simulink model "Barriere_fermeture_geometrique_2016a"  (R2016b)
settings: Solver=VariableStepAuto  StartTime=0.0  StopTime=10.0  RelTol=1e-3
PreLoadFcn:
  | addpath('Simscape')
model workspace (MATLAB code in the model file):
  | % Simscape(TM) Multibody(TM) version: 7.0
  | 
  | % This is a model data file derived from a Simscape Multibody Import XML file using the smimport function.
  | % The data in this file sets the block parameter values in an imported Simscape Multibody model.
  | % For more information on this file, see the smimport function help page in the Simscape Multibody documentation.
  | % You can modify numerical values, but avoid any other changes to this file.
  | % Do not add code to this file. Do not edit the physical units shown in comments.
  | 
  | %%%VariableName:smiData
  | 
  | 
  | %============= RigidTransform =============%
  | 
  | %Initialize the RigidTransform structure array by filling in null values.
  | smiData.RigidTransform(115).translation = [0.0 0.0 0.0];
  | smiData.RigidTransform(115).angle = 0.0;
  | smiData.RigidTransform(115).axis = [0.0 0.0 0.0];
  | smiData.RigidTransform(115).ID = '';
  | 
  | %Translation Method - Cartesian
  | %Rotation Method - Arbitrary Axis
  | smiData.RigidTransform(1).translation = [0 0 0];  % mm
  | smiData.RigidTransform(1).angle = 0;  % rad
  | smiData.RigidTransform(1).axis = [0 0 0];
  | smiData.RigidTransform(1).ID = 'B[Bati-1:-:]';
  | 
  | %Translation Method - Cartesian
  | %Rotation Method - Arbitrary Axis
  | smiData.RigidTransform(2).translation = [0 0 0];  % mm
  | smiData.RigidTransform(2).angle = 0;  % rad
  | smiData.RigidTransform(2).axis = [0 0 0];
  | smiData.RigidTransform(2).ID = 'F[Bati-1:-:]';
  | 
  | %Translation Method - Cartesian
  | %Rotation Method - Arbitrary Axis
  | smiData.RigidTransform(3).translation = [-1.4921397450962104e-13 -2.1187831252329945e-13 201.81368327358359];  % mm
  | smiData.RigidTransform(3).angle = 2.0943951023931962;  % rad
  | smiData.RigidTransform(3).axis = [0.57735026918962606 -0.57735026918962595 0.5773502691896254];
  | smiData.RigidTransform(3).ID = 'B[Bati-1:-:Manivelle-1]';
  | 
  | %Translation Method - Cartesian
  | %Rotation Method - Arbitrary Axis
  | smiData.RigidTransform(4).translation = [-1.4110480386564174e-11 -34.999999999999446 1.9203073623444143e-11];  % mm
  | smiData.RigidTransform(4).angle = 2.0943951023931944;  % rad
  | smiData.RigidTransform(4).axis = [-0.57735026918962551 -0.57735026918962451 -0.57735026918962729];
  | smiData.RigidTransform(4).ID = 'F[Bati-1:-:Manivelle-1]';
  | 
  | %Translation Method - Cartesian
  | %Rotation Method - Arbitrary Axis
  | smiData.RigidTransform(5).translation = [79.008796978564504 9.0000000000000036 -5.500000000000286];  % mm
  | smiData.RigidTransform(5).angle = 2.0943951023931966;  % rad
  | smiData.RigidTransform(5).axis = [0.57735026918962606 -0.57735026918962595 0.57735026918962529];
  | smiData.RigidTransform(5).ID = 'B[Manivelle-1:-:Roue-1]';
  | 
  | %Translation Method - Cartesian
  | %Rotation Method - Arbitrary Axis
  | smiData.RigidTransform(6).translation = [1.0096423697092405e-11 1.4694134797821334e-11 -1.0000000000000713];  % mm
  | smiData.RigidTransform(6).angle = 3.1415926535897931;  % rad
  | smiData.RigidTransform(6).axis = [1 -3.6232584844029224e-34 -2.1942087839562885e-16];
  | smiData.RigidTransform(6).ID = 'F[Manivelle-1:-:Roue-1]';
  | 
  | %Translation Method - Cartesian
  | %Rotation Method - Arbitrary Axis
  | smiData.RigidTransform(7).translation = [2.4950194972320238e-13 126.79563556224846 92.813683273583734];  % mm
  | smiData.RigidTransform(7).angle = 2.0943951023931962;  % rad
  | smiData.RigidTransform(7).axis = [0.57735026918962606 -0.57735026918962529 0.57735026918962606];
  | smiData.RigidTransform(7).ID = 'B[Bati-1:-:Bielle-1]';
  | 
  | %Translation Method - Cartesian
  | %Rotation Method - Arbitrary Axis
  | smiData.RigidTransform(8).translation = [-1.33896240562668e-12 -185.69563556224858 1.7011796269739942e-14];  % mm
  | smiData.RigidTransform(8).angle = 2.0943951023931962;  % rad
  | smiData.RigidTransform(8).axis = [-0.57735026918962606 -0.57735026918962606 -0.57735026918962529];
  | smiData.RigidTransform(8).ID = 'F[Bati-1:-:Bielle-1]';
  | 
  | %Translation Method - Cartesian
  | %Rotation Method - Arbitrary Axis
  | smiData.RigidTransform(9).translation = [-132.59544790787075 -8.5265128291212022e-14 146.46653950343381];  % mm
  | smiData.RigidTransform(9).angle = 3.1415926535897931;  % rad
  | smiData.RigidTransform(9).axis = [-0.92883739768533258 -1.4174241145510651e-17 0.37048763631346637];
  | smiData.RigidTransform(9).ID = 'B[Bielle-1:-:Roue-1]';
  | 
  | %Translation Method - Cartesian
  | %Rotation Method - Arbitrary Axis
  | smiData.RigidTransform(10).translation = [-73.757110325617248 103.72960409807774 13.900000000000148];  % mm
  | smiData.RigidTransform(10).angle = 1.8341255936563658;  % rad
  | smiData.RigidTransform(10).axis = [-0.76611237185348935 0.45446222818459925 -0.45446222818459875];
  | smiData.RigidTransform(10).ID = 'F[Bielle-1:-:Roue-1]';
  | 
  | %Translation Method - Cartesian
  | %Rotation Method - Arbitrary Axis
  | smiData.RigidTransform(11).translation = [-855.00000000000057 -415.99999999999989 -2.997602166487909e-13];  % mm
  | smiData.RigidTransform(11).angle = 2.0943951023931953;  % rad
  | smiData.RigidTransform(11).axis = [0.57735026918962584 0.57735026918962562 0.57735026918962584];
  | smiData.RigidTransform(11).ID = 'B[Bielle-1:-:Masse_mobile-1]';
  | 
  | %Translation Method - Cartesian
  | %Rotation Method - Arbitrary Axis
  | smiData.RigidTransform(12).translation = [1155.7022886337502 2.6435895478936817e-14 1.7053025658242339e-13];  % mm
  | smiData.RigidTransform(12).angle = 2.0943951023931953;  % rad
  | smiData.RigidTransform(12).axis = [-0.57735026918962584 -0.57735026918962584 0.57735026918962584];
  | smiData.RigidTransform(12).ID = 'F[Bielle-1:-:Masse_mobile-1]';
  | 
  | %Translation Method - Cartesian
  | %Rotation Method - Arbitrary Axis
  | smiData.RigidTransform(13).translation = [0 0 43.813683273583607];  % mm
  | smiData.RigidTransform(13).angle = 3.1415926535897931;  % rad
  | smiData.RigidTransform(13).axis = [0 -7.6859349917756591e-17 1];
  | smiData.RigidTransform(13).ID = 'AssemblyGround[Bati-1:3742-1]';
  | 
  | %Translation Method - Cartesian
  | %Rotation Method - Arbitrary Axis
  | smiData.RigidTransform(14).translation = [124.99999999999996 229.50000000000017 49.813683273583663];  % mm
  | smiData.RigidTransform(14).angle = 1.8025643331517374;  % rad
  | smiData.RigidTransform(14).axis = [6.4891737650865717e-17 -5.7309259263021267e-17 1];
  | smiData.RigidTransform(14).ID = 'AssemblyGround[Bati-1:eh_12-1]';
  | 
  | %Translation Method - Cartesian
  | %Rotation Method - Arbitrary Axis
  | smiData.RigidTransform(15).translation = [-175.8775777875249 210.38468501103969 136.63945712062966];  % mm
  | smiData.RigidTransform(15).angle = 1.6861590425374564;  % rad
  | smiData.RigidTransform(15).axis = [0.5173147433723283 0.79319630861479418 0.32128658902837226];
  | smiData.RigidTransform(15).ID = 'AssemblyGround[Bati-1:Moteur-1:ehfr_6-1]';
  | 
  | %Translation Method - Cartesian
  | %Rotation Method - Arbitrary Axis
  | smiData.RigidTransform(16).translation = [-194.42155942355888 175.34681984943683 174.99999999999707];  % mm
  | smiData.RigidTransform(16).angle = 1.9203799458038229;  % rad
  | smiData.RigidTransform(16).axis = [0.36625265461228562 0.28987567884942211 -0.88421212602013133];
  | smiData.RigidTransform(16).ID = 'AssemblyGround[Bati-1:Moteur-1:MOTEUR_014-1]';
  | 
  | %Translation Method - Cartesian
  | %Rotation Method - Arbitrary Axis
  | smiData.RigidTransform(17).translation = [-175.87757778752552 210.38468501103691 213.36054287936705];  % mm
  | smiData.RigidTransform(17).angle = 1.6861590425374564;  % rad
  | smiData.RigidTransform(17).axis = [0.5173147433723283 0.79319630861479418 0.32128658902837226];
  | smiData.RigidTransform(17).ID = 'AssemblyGround[Bati-1:Moteur-1:ehfr_6-2]';
  | 
  | %Translation Method - Cartesian
  | %Rotation Method - Arbitrary Axis
  | smiData.RigidTransform(18).translation = [-193.50030490480947 135.71498239378184 213.36054287937054];  % mm
  | smiData.RigidTransform(18).angle = 1.5798154611582129;  % rad
  | smiData.RigidTransform(18).axis = [0.13562103621123053 0.98623959459989585 -0.094543093774347442];
  | smiData.RigidTransform(18).ID = 'AssemblyGround[Bati-1:Moteur-1:ehfr_6-3]';
  | 
  | %Translation Method - Cartesian
  | %Rotation Method - Arbitrary Axis
  | smiData.RigidTransform(19).translation = [-189.50324309587222 213.6004656168802 136.63945712062966];  % mm
  | smiData.RigidTransform(19).angle = 2.682320000710968;  % rad
  | smiData.RigidTransform(19).axis = [0.61543871803223826 -0.38543093102275494 -0.68751595018426104];
  | smiData.RigidTransform(19).ID = 'AssemblyGround[Bati-1:Moteur-1:vchc_6_30-1]';
  | 
  | %Translation Method - Cartesian
  | %Rotation Method - Arbitrary Axis
  | smiData.RigidTransform(20).translation = [-207.12597021315676 138.93076299962223 136.63945712062986];  % mm
  | smiData.RigidTransform(20).angle = 2.4395162248310025;  % rad
  | smiData.RigidTransform(20).axis = [0.55627663095078395 -0.50755250127944629 -0.65798690587505093];
  | smiData.RigidTransform(20).ID = 'AssemblyGround[Bati-1:Moteur-1:vchc_6_30-2]';
  | 
  | %Translation Method - Cartesian
  | %Rotation Method - Arbitrary Axis
  | smiData.RigidTransform(21).translation = [-207.12597021315671 138.93076299962235 213.36054287937054];  % mm
  | smiData.RigidTransform(21).angle = 2.4395162248310025;  % rad
  | smiData.RigidTransform(21).axis = [0.55627663095078395 -0.50755250127944629 -0.65798690587505093];
  | smiData.RigidTransform(21).ID = 'AssemblyGround[Bati-1:Moteur-1:vchc_6_30-3]';
  | 
  | %Translation Method - Cartesian
  | %Rotation Method - Arbitrary Axis
  | smiData.RigidTransform(22).translation = [-189.50324309587285 213.60046561687741 213.36054287936705];  % mm
  | smiData.RigidTransform(22).angle = 2.4395162248310025;  % rad
  | smiData.RigidTransform(22).axis = [0.55627663095078395 -0.50755250127944629 -0.65798690587505093];
  | smiData.RigidTransform(22).ID = 'AssemblyGround[Bati-1:Moteur-1:vchc_6_30-4]';
  | 
  | %Translation Method - Cartesian
  | %Rotation Method - Arbitrary Axis
  | smiData.RigidTransform(23).translation = [-193.50030490480938 135.71498239378172 136.63945712062986];  % mm
  | smiData.RigidTransform(23).angle = 1.5798154611582129;  % rad
  | smiData.RigidTransform(23).axis = [0.13562103621123026 0.98623959459989607 -0.094543093774347456];
  | smiData.RigidTransform(23).ID = 'AssemblyGround[Bati-1:Moteur-1:ehfr_6-4]';
  | 
  | %Translation Method - Cartesian
  | %Rotation Method - Arbitrary Axis
  | smiData.RigidTransform(24).translation = [125.99999999999656 229.50000000000006 46.813683273586562];  % mm
  | smiData.RigidTransform(24).angle = 1.8025643331517369;  % rad
  | smiData.RigidTransform(24).axis = [6.3930876709235808e-17 -1.1805373058737908e-16 1];
  | smiData.RigidTransform(24).ID = 'AssemblyGround[Bati-1:Moteur-1]';
  | 
  | %Translation Method - Cartesian
  | %Rotation Method - Arbitrary Axis
  | smiData.RigidTransform(25).translation = [64.223317737885779 178.52133054270737 21.000000000000053];  % mm
  | smiData.RigidTransform(25).angle = 1.3390283204380566;  % rad
  | smiData.RigidTransform(25).axis = [1.3951389385649892e-16 -1.4208309664535837e-16 1];
  | smiData.RigidTransform(25).ID = 'AssemblyGround[Bati-1:Roulement_2-1:ehfr_14-2]';
  | 
  | %Translation Method - Cartesian
  | %Rotation Method - Arbitrary Axis
  | smiData.RigidTransform(26).translation = [64.223317737885779 178.52133054270737 19.000000000000053];  % mm
  | smiData.RigidTransform(26).angle = 1.3390283204380566;  % rad
  | smiData.RigidTransform(26).axis = [1.3951389385649892e-16 -1.4208309664535837e-16 1];
  | smiData.RigidTransform(26).ID = 'AssemblyGround[Bati-1:Roulement_2-1:rond_m_14-2]';
  | 
  | %Translation Method - Cartesian
  | %Rotation Method - Arbitrary Axis
  | smiData.RigidTransform(27).translation = [64.223317737885779 178.52133054270737 -5.9999999999999565];  % mm
  | smiData.RigidTransform(27).angle = 1.586709603785015;  % rad
  | smiData.RigidTransform(27).axis = [0.98421200917482088 -0.12515334792977473 -0.12515334792977512];
  | smiData.RigidTransform(27).ID = 'AssemblyGround[Bati-1:Roulement_2-1:VIS_TF2E_001-2]';
  | 
  | %Translation Method - Cartesian
  | %Rotation Method - Arbitrary Axis
  | smiData.RigidTransform(28).translation = [35.051593670618466 54.91708095984221 21.000000000000011];  % mm
  | smiData.RigidTransform(28).angle = 1.3390283204380566;  % rad
  | smiData.RigidTransform(28).axis = [1.3951389385649892e-16 -1.4208309664535837e-16 1];
  | smiData.RigidTransform(28).ID = 'AssemblyGround[Bati-1:Roulement_2-1:ehfr_14-1]';
  | 
  | %Translation Method - Cartesian
  | %Rotation Method - Arbitrary Axis
  | smiData.RigidTransform(29).translation = [49.637455704252211 116.719205751275 0];  % mm
  | smiData.RigidTransform(29).angle = 1.8025643331517369;  % rad
  | smiData.RigidTransform(29).axis = [9.3810881603968918e-17 2.516618558763085e-16 -1];
  | smiData.RigidTransform(29).ID = 'AssemblyGround[Bati-1:Roulement_2-1:roul_010-1]';
  | 
  | %Translation Method - Cartesian
  | %Rotation Method - Arbitrary Axis
  | smiData.RigidTransform(30).translation = [35.051593670618466 54.91708095984221 19.000000000000011];  % mm
  | smiData.RigidTransform(30).angle = 1.3390283204380566;  % rad
  | smiData.RigidTransform(30).axis = [1.3951389385649892e-16 -1.4208309664535837e-16 1];
  | smiData.RigidTransform(30).ID = 'AssemblyGround[Bati-1:Roulement_2-1:rond_m_14-1]';
  | 
  | %Translation Method - Cartesian
  | %Rotation Method - Arbitrary Axis
  | smiData.RigidTransform(31).translation = [35.051593670618466 54.917080959842238 -5.9999999999998526];  % mm
  | smiData.RigidTransform(31).angle = 1.584165821206561;  % rad
  | smiData.RigidTransform(31).axis = [0.98671908730881319 -0.11485957239268889 -0.114859572392689];
  | smiData.RigidTransform(31).ID = 'AssemblyGround[Bati-1:Roulement_2-1:VIS_TF2E_001-1]';
  | 
  | %Translation Method - Cartesian
  | %Rotation Method - Arbitrary Axis
  | smiData.RigidTransform(32).translation = [124.81984509590156 230.00190937854114 49.813683273583685];  % mm
  | smiData.RigidTransform(32).angle = 1.8025643331517369;  % rad
  | smiData.RigidTransform(32).axis = [-9.3810881603968918e-17 -2.516618558763085e-16 1];
  | smiData.RigidTransform(32).ID = 'AssemblyGround[Bati-1:Roulement_2-1]';
  | 
  | %Translation Method - Cartesian
  | %Rotation Method - Arbitrary Axis
  | smiData.RigidTransform(33).translation = [124.99999999999994 21.00000000000005 49.813683273583685];  % mm
  | smiData.RigidTransform(33).angle = 1.8025643331517374;  % rad
  | smiData.RigidTransform(33).axis = [6.4891737650865717e-17 -5.7309259263021267e-17 1];
  | smiData.RigidTransform(33).ID = 'AssemblyGround[Bati-1:eh_12-2]';
  | 
  | %Translation Method - Cartesian
  | %Rotation Method - Arbitrary Axis
  | smiData.RigidTransform(34).translation = [-125 229.50000000000017 49.813683273583656];  % mm
  | smiData.RigidTransform(34).angle = 1.8025643331517374;  % rad
  | smiData.RigidTransform(34).axis = [6.4891737650865717e-17 -5.7309259263021267e-17 1];
  | smiData.RigidTransform(34).ID = 'AssemblyGround[Bati-1:eh_12-3]';
  | 
  | %Translation Method - Cartesian
  | %Rotation Method - Arbitrary Axis
  | smiData.RigidTransform(35).translation = [-125.00000000000006 21.000000000000046 49.813683273583699];  % mm
  | smiData.RigidTransform(35).angle = 1.8025643331517374;  % rad
  | smiData.RigidTransform(35).axis = [0 0 1];
  | smiData.RigidTransform(35).ID = 'AssemblyGround[Bati-1:eh_12-4]';
  | 
  | %Translation Method - Cartesian
  | %Rotation Method - Arbitrary Axis
  | smiData.RigidTransform(36).translation = [-233.39343399959662 123.4099062712389 43.000000000000028];  % mm
  | smiData.RigidTransform(36).angle = 2.1269062011022761;  % rad
  | smiData.RigidTransform(36).axis = [-0.44439290189209107 0.67602805443717784 -0.58779334664643024];
  | smiData.RigidTransform(36).ID = 'AssemblyGround[Bati-1:Roulement_1-1:rond_m_10-2]';
  | 
  | %Translation Method - Cartesian
  | %Rotation Method - Arbitrary Axis
  | smiData.RigidTransform(37).translation = [-205.93473899471468 237.14371860789134 43.000000000000057];  % mm
  | smiData.RigidTransform(37).angle = 3.0234649588732694;  % rad
  | smiData.RigidTransform(37).axis = [-0.70057844934475677 0.10458570654058162 0.70586943998242579];
  | smiData.RigidTransform(37).ID = 'AssemblyGround[Bati-1:Roulement_1-1:vh_10_45 8-8-1]';
  | 
  | %Translation Method - Cartesian
  | %Rotation Method - Arbitrary Axis
  | smiData.RigidTransform(38).translation = [-231.44691038411835 122.9505090418331 43.000000000000028];  % mm
  | smiData.RigidTransform(38).angle = 1.8561332144596066;  % rad
  | smiData.RigidTransform(38).axis = [0.6281370768124086 0.62112083286202469 0.46867123201488148];
  | smiData.RigidTransform(38).ID = 'AssemblyGround[Bati-1:Roulement_1-1:ENTRETOISE_023-2]';
  | 
  | %Translation Method - Cartesian
  | %Rotation Method - Arbitrary Axis
  | smiData.RigidTransform(39).translation = [-204.38387611565184 176.67054418872968 43.000000000000043];  % mm
  | smiData.RigidTransform(39).angle = 2.2329912010448152;  % rad
  | smiData.RigidTransform(39).axis = [0.48837040813325044 -0.6170471393904029 -0.6170471393904059];
  | smiData.RigidTransform(39).ID = 'AssemblyGround[Bati-1:Roulement_1-1:roul_009-1]';
  | 
  | %Translation Method - Cartesian
  | %Rotation Method - Arbitrary Axis
  | smiData.RigidTransform(40).translation = [-232.80947691495311 123.27208710241713 43.000000000000028];  % mm
  | smiData.RigidTransform(40).angle = 3.0234649588732694;  % rad
  | smiData.RigidTransform(40).axis = [-0.70057844934475666 0.10458570654058141 0.70586943998242591];
  | smiData.RigidTransform(40).ID = 'AssemblyGround[Bati-1:Roulement_1-1:vh_10_45 8-8-2]';
  | 
  | %Translation Method - Cartesian
  | %Rotation Method - Arbitrary Axis
  | smiData.RigidTransform(41).translation = [-204.57217246387992 236.82214054730727 43.000000000000057];  % mm
  | smiData.RigidTransform(41).angle = 2.232991201044813;  % rad
  | smiData.RigidTransform(41).axis = [-0.48837040813324945 0.61704713939040501 -0.61704713939040456];
  | smiData.RigidTransform(41).ID = 'AssemblyGround[Bati-1:Roulement_1-1:ENTRETOISE_023-1]';
  | 
  | %Translation Method - Cartesian
  | %Rotation Method - Arbitrary Axis
  | smiData.RigidTransform(42).translation = [-202.24905615194552 116.05955060074632 43.000000000000028];  % mm
  | smiData.RigidTransform(42).angle = 1.5777653498429955;  % rad
  | smiData.RigidTransform(42).axis = [0.14713680523855655 0.98561149764352873 -0.083190962592528811];
  | smiData.RigidTransform(42).ID = 'AssemblyGround[Bati-1:Roulement_1-1:ehfr_10-2]';
  | 
  | %Translation Method - Cartesian
  | %Rotation Method - Arbitrary Axis
  | smiData.RigidTransform(43).translation = [-175.37431823170709 229.93118210622052 43.000000000000057];  % mm
  | smiData.RigidTransform(43).angle = 2.3554366301540348;  % rad
  | smiData.RigidTransform(43).axis = [-0.53100028324755 0.55137024942272572 -0.64345127806427027];
  | smiData.RigidTransform(43).ID = 'AssemblyGround[Bati-1:Roulement_1-1:ehfr_10-1]';
  | 
  | %Translation Method - Cartesian
  | %Rotation Method - Arbitrary Axis
  | smiData.RigidTransform(44).translation = [-206.51869607935814 237.28153777671307 43.000000000000057];  % mm
  | smiData.RigidTransform(44).angle = 3.1212647204710873;  % rad
  | smiData.RigidTransform(44).axis = [0.69049920252183583 -0.15252051659504276 0.70707025346445607];
  | smiData.RigidTransform(44).ID = 'AssemblyGround[Bati-1:Roulement_1-1:rond_m_10-1]';
  | 
  | %Translation Method - Cartesian
  | %Rotation Method - Arbitrary Axis
  | smiData.RigidTransform(45).translation = [125.00000000000017 229.50000000000017 49.813683273583898];  % mm
  | smiData.RigidTransform(45).angle = 1.8025643331517378;  % rad
  | smiData.RigidTransform(45).axis = [-2.9335469981929225e-16 -2.9342350937782738e-16 1];
  | smiData.RigidTransform(45).ID = 'AssemblyGround[Bati-1:Roulement_1-1]';
  | 
  | %Translation Method - Cartesian
  | %Rotation Method - Arbitrary Axis
  | smiData.RigidTransform(46).translation = [-125 229.5 43.813683273583777];  % mm
  | smiData.RigidTransform(46).angle = 3.1415926535897931;  % rad
  | smiData.RigidTransform(46).axis = [-0.98074665978199183 -0.1952843806515665 -1.3884606460031711e-16];
  | smiData.RigidTransform(46).ID = 'AssemblyGround[Bati-1:entretoise base-1]';
  | 
  | %Translation Method - Cartesian
  | %Rotation Method - Arbitrary Axis
  | smiData.RigidTransform(47).translation = [124.99999999999999 21.000000000000043 43.813683273583727];  % mm
  | smiData.RigidTransform(47).angle = 3.1415926535897931;  % rad
  | smiData.RigidTransform(47).axis = [-0.98074665978199183 -0.1952843806515665 -1.3884606460031711e-16];
  | smiData.RigidTransform(47).ID = 'AssemblyGround[Bati-1:entretoise base-4]';
  | 
  | %Translation Method - Cartesian
  | %Rotation Method - Arbitrary Axis
  | smiData.RigidTransform(48).translation = [0 0 0];  % mm
  | smiData.RigidTransform(48).angle = 1.5707963267948968;  % rad
  | smiData.RigidTransform(48).axis = [1 0 0];
  | smiData.RigidTransform(48).ID = 'AssemblyGround[Bati-1:support moteur-1]';
  | 
  | %Translation Method - Cartesian
  | %Rotation Method - Arbitrary Axis
  | smiData.RigidTransform(49).translation = [-160.0000000000004 -287.99999999999989 -10.000000000000002];  % mm
  | smiData.RigidTransform(49).angle = 2.0943951023931953;  % rad
  | smiData.RigidTransform(49).axis = [-0.57735026918962595 -0.57735026918962562 0.57735026918962562];
  | smiData.RigidTransform(49).ID = 'AssemblyGround[Bati-1:pied-1:plateau superieur-1]';
  | 
  | %Translation Method - Cartesian
  | %Rotation Method - Arbitrary Axis
  | smiData.RigidTransform(50).translation = [-125.00000000000189 -200.50000000000304 -912.9999999999925];  % mm
  | smiData.RigidTransform(50).angle = 1.5707963267948968;  % rad
  | smiData.RigidTransform(50).axis = [1 -1.6431300764452314e-14 0];
  | smiData.RigidTransform(50).ID = 'AssemblyGround[Bati-1:pied-1:base pied-1]';
  | 
  | %Translation Method - Cartesian
  | %Rotation Method - Arbitrary Axis
  | smiData.RigidTransform(51).translation = [-474.99999999997806 -300.500000000005 -920.9999999999925];  % mm
  | smiData.RigidTransform(51).angle = 1.5707963267948968;  % rad
  | smiData.RigidTransform(51).axis = [1 0 0];
  | smiData.RigidTransform(51).ID = 'AssemblyGround[Bati-1:pied-1:socle-1]';
  | 
  | %Translation Method - Cartesian
  | %Rotation Method - Arbitrary Axis
  | smiData.RigidTransform(52).translation = [-125.00000000000028 -122.50000000000315 -912.9999999999925];  % mm
  | smiData.RigidTransform(52).angle = 2.0943951023931859;  % rad
  | smiData.RigidTransform(52).axis = [0.57735026918962262 -0.57735026918963206 0.57735026918962262];
  | smiData.RigidTransform(52).ID = 'AssemblyGround[Bati-1:pied-1:renfort pied-1]';
  | 
  | %Translation Method - Cartesian
  | %Rotation Method - Arbitrary Axis
  | smiData.RigidTransform(53).translation = [0 0 43.813683273583877];  % mm
  | smiData.RigidTransform(53).angle = 3.1415926535897927;  % rad
  | smiData.RigidTransform(53).axis = [-0 -0 -1];
  | smiData.RigidTransform(53).ID = 'AssemblyGround[Bati-1:pied-1]';
  | 
  | %Translation Method - Cartesian
  | %Rotation Method - Arbitrary Axis
  | smiData.RigidTransform(54).translation = [136.49999999999997 256 -50];  % mm
  | smiData.RigidTransform(54).angle = 1.5707963267948968;  % rad
  | smiData.RigidTransform(54).axis = [1 0 0];
  | smiData.RigidTransform(54).ID = 'AssemblyGround[Bati-1:Assemblage pupitre-1:C60-1]';
  | 
  | %Translation Method - Cartesian
  | %Rotation Method - Arbitrary Axis
  | smiData.RigidTransform(55).translation = [122.00000000000001 88.999999999999972 3.5000000000000031];  % mm
  | smiData.RigidTransform(55).angle = 2.8645335361772575;  % rad
  | smiData.RigidTransform(55).axis = [0.13942256184718882 -0.70020045317322044 -0.70020045317322044];
  | smiData.RigidTransform(55).ID = 'AssemblyGround[Bati-1:Assemblage pupitre-1:douille_4mm_rouge-1]';
  | 
  | %Translation Method - Cartesian
  | %Rotation Method - Arbitrary Axis
  | smiData.RigidTransform(56).translation = [182 70 3.5000000000000031];  % mm
  | smiData.RigidTransform(56).angle = 2.8645335361772575;  % rad
  | smiData.RigidTransform(56).axis = [0.13942256184718882 -0.70020045317322044 -0.70020045317322044];
  | smiData.RigidTransform(56).ID = 'AssemblyGround[Bati-1:Assemblage pupitre-1:douille_4mm_rouge-5]';
  | 
  | %Translation Method - Cartesian
  | %Rotation Method - Arbitrary Axis
  | smiData.RigidTransform(57).translation = [102.49999999999997 110.49999999999993 10.500000000000002];  % mm
  | smiData.RigidTransform(57).angle = 0;  % rad
  | smiData.RigidTransform(57).axis = [0 0 0];
  | smiData.RigidTransform(57).ID = 'AssemblyGround[Bati-1:Assemblage pupitre-1:atv-1]';
  | 
  | %Translation Method - Cartesian
  | %Rotation Method - Arbitrary Axis
  | smiData.RigidTransform(58).translation = [152 88.999999999999972 3.5000000000000031];  % mm
  | smiData.RigidTransform(58).angle = 2.8645335361772575;  % rad
  | smiData.RigidTransform(58).axis = [0.13942256184718882 -0.70020045317322044 -0.70020045317322044];
  | smiData.RigidTransform(58).ID = 'AssemblyGround[Bati-1:Assemblage pupitre-1:douille_4mm_rouge-4]';
  | 
  | %Translation Method - Cartesian
  | %Rotation Method - Arbitrary Axis
  | smiData.RigidTransform(59).translation = [182 89.000000000000028 3.5000000000000031];  % mm
  | smiData.RigidTransform(59).angle = 2.8645335361772575;  % rad
  | smiData.RigidTransform(59).axis = [0.13942256184718882 -0.70020045317322044 -0.70020045317322044];
  | smiData.RigidTransform(59).ID = 'AssemblyGround[Bati-1:Assemblage pupitre-1:douille_4mm_rouge-2]';
  | 
  | %Translation Method - Cartesian
  | %Rotation Method - Arbitrary Axis
  | smiData.RigidTransform(60).translation = [122.00000000000003 69.999999999999957 3.5000000000000031];  % mm
  | smiData.RigidTransform(60).angle = 2.8645335361772575;  % rad
  | smiData.RigidTransform(60).axis = [0.13942256184718882 -0.70020045317322044 -0.70020045317322044];
  | smiData.RigidTransform(60).ID = 'AssemblyGround[Bati-1:Assemblage pupitre-1:douille_4mm_rouge-3]';
  | 
  | %Translation Method - Cartesian
  | %Rotation Method - Arbitrary Axis
  | smiData.RigidTransform(61).translation = [15 15 -20.000000000000018];  % mm
  | smiData.RigidTransform(61).angle = 0;  % rad
  | smiData.RigidTransform(61).axis = [0 0 0];
  | smiData.RigidTransform(61).ID = 'AssemblyGround[Bati-1:Assemblage pupitre-1:bouton_tournant_clé-1:embase_BT_clé-2]';
  | 
  | %Translation Method - Cartesian
  | %Rotation Method - Arbitrary Axis
  | smiData.RigidTransform(62).translation = [12.483450518527395 35.01481477798076 -21.990742270930674];  % mm
  | smiData.RigidTransform(62).angle = 1.0104350246787706;  % rad
  | smiData.RigidTransform(62).axis = [-0.0054592338395522983 -0.999968069200867 -0.0058358670799844572];
  | smiData.RigidTransform(62).ID = 'AssemblyGround[Bati-1:Assemblage pupitre-1:bouton_tournant_clé-1:clé-1]';
  | 
  | %Translation Method - Cartesian
  | %Rotation Method - Arbitrary Axis
  | smiData.RigidTransform(63).translation = [0 0 0];  % mm
  | smiData.RigidTransform(63).angle = 0;  % rad
  | smiData.RigidTransform(63).axis = [0 0 0];
  | smiData.RigidTransform(63).ID = 'AssemblyGround[Bati-1:Assemblage pupitre-1:bouton_tournant_clé-1:embase_BP_2_contacts-1]';
  | 
  | %Translation Method - Cartesian
  | %Rotation Method - Arbitrary Axis
  | smiData.RigidTransform(64).translation = [15 24.000000000000007 -20.000000000000018];  % mm
  | smiData.RigidTransform(64).angle = 0;  % rad
  | smiData.RigidTransform(64).axis = [0 0 0];
  | smiData.RigidTransform(64).ID = 'AssemblyGround[Bati-1:Assemblage pupitre-1:bouton_tournant_clé-1:corps_BT_clé-1]';
  | 
  | %Translation Method - Cartesian
  | %Rotation Method - Arbitrary Axis
  | smiData.RigidTransform(65).translation = [22.000000000000007 94.999999999999972 -13.500000000000012];  % mm
  | smiData.RigidTransform(65).angle = 1.5707963267948968;  % rad
  | smiData.RigidTransform(65).axis = [1 0 0];
  | smiData.RigidTransform(65).ID = 'AssemblyGround[Bati-1:Assemblage pupitre-1:bouton_tournant_clé-1]';
  | 
  | %Translation Method - Cartesian
  | %Rotation Method - Arbitrary Axis
  | smiData.RigidTransform(66).translation = [-8.0000000000000071 0 0];  % mm
  | smiData.RigidTransform(66).angle = 0;  % rad
  | smiData.RigidTransform(66).axis = [0 0 0];
  | smiData.RigidTransform(66).ID = 'AssemblyGround[Bati-1:Assemblage pupitre-1:tole mesures-1]';
  | 
  | %Translation Method - Cartesian
  | %Rotation Method - Arbitrary Axis
  | smiData.RigidTransform(67).translation = [0 0 21.999999999999993];  % mm
  | smiData.RigidTransform(67).angle = 0;  % rad
  | smiData.RigidTransform(67).axis = [0 0 0];
  | smiData.RigidTransform(67).ID = 'AssemblyGround[Bati-1:Assemblage pupitre-1:voyant_vert-1:tête_voyant_vert-1]';
  | 
  | %Translation Method - Cartesian
  | %Rotation Method - Arbitrary Axis
  | smiData.RigidTransform(68).translation = [0 0 0];  % mm
  | smiData.RigidTransform(68).angle = 0;  % rad
  | smiData.RigidTransform(68).axis = [0 0 0];
  | smiData.RigidTransform(68).ID = 'AssemblyGround[Bati-1:Assemblage pupitre-1:voyant_vert-1:corps_voyant_24V-1]';
  | 
  | %Translation Method - Cartesian
  | %Rotation Method - Arbitrary Axis
  | smiData.RigidTransform(69).translation = [37.000000000000007 305.00000000000006 -20.499999999999989];  % mm
  | smiData.RigidTransform(69).angle = 0;  % rad
  | smiData.RigidTransform(69).axis = [0 0 0];
  | smiData.RigidTransform(69).ID = 'AssemblyGround[Bati-1:Assemblage pupitre-1:voyant_vert-1]';
  | 
  | %Translation Method - Cartesian
  | %Rotation Method - Arbitrary Axis
  | smiData.RigidTransform(70).translation = [152 69.999999999999957 3.5000000000000031];  % mm
  | smiData.RigidTransform(70).angle = 2.8645335361772575;  % rad
  | smiData.RigidTransform(70).axis = [0.13942256184718882 -0.70020045317322044 -0.70020045317322044];
  | smiData.RigidTransform(70).ID = 'AssemblyGround[Bati-1:Assemblage pupitre-1:douille_4mm_rouge-6]';
  | 
  | %Translation Method - Cartesian
  | %Rotation Method - Arbitrary Axis
  | smiData.RigidTransform(71).translation = [-1.999999999999988 -17.999999999999989 24.999999999999996];  % mm
  | smiData.RigidTransform(71).angle = 0;  % rad
  | smiData.RigidTransform(71).axis = [0 0 0];
  | smiData.RigidTransform(71).ID = 'AssemblyGround[Bati-1:Assemblage pupitre-1:inter_sectionneur-1:inter_sectionneur_vario_4-1]';
  | 
  | %Translation Method - Cartesian
  | %Rotation Method - Arbitrary Axis
  | smiData.RigidTransform(72).translation = [0 0 0];  % mm
  | smiData.RigidTransform(72).angle = 0;  % rad
  | smiData.RigidTransform(72).axis = [0 0 0];
  | smiData.RigidTransform(72).ID = 'AssemblyGround[Bati-1:Assemblage pupitre-1:inter_sectionneur-1:inter_sectionneur_vario_1-1]';
  | 
  | %Translation Method - Cartesian
  | %Rotation Method - Arbitrary Axis
  | smiData.RigidTransform(73).translation = [0 0 0];  % mm
  | smiData.RigidTransform(73).angle = 0;  % rad
  | smiData.RigidTransform(73).axis = [0 0 0];
  | smiData.RigidTransform(73).ID = 'AssemblyGround[Bati-1:Assemblage pupitre-1:inter_sectionneur-1:inter_sectionneur_vario_2-1]';
  | 
  | %Translation Method - Cartesian
  | %Rotation Method - Arbitrary Axis
  | smiData.RigidTransform(74).translation = [0 0 -0.50000000000000044];  % mm
  | smiData.RigidTransform(74).angle = 0;  % rad
  | smiData.RigidTransform(74).axis = [0 0 0];
  | smiData.RigidTransform(74).ID = 'AssemblyGround[Bati-1:Assemblage pupitre-1:inter_sectionneur-1:inter_sectionneur_vario_3-1]';
  | 
  | %Translation Method - Cartesian
  | %Rotation Method - Arbitrary Axis
  | smiData.RigidTransform(75).translation = [36.999999999999993 240 1.5000000000000013];  % mm
  | smiData.RigidTransform(75).angle = 0;  % rad
  | smiData.RigidTransform(75).axis = [0 0 0];
  | smiData.RigidTransform(75).ID = 'AssemblyGround[Bati-1:Assemblage pupitre-1:inter_sectionneur-1]';
  | 
  | %Translation Method - Cartesian
  | %Rotation Method - Arbitrary Axis
  | smiData.RigidTransform(76).translation = [122.00000000000001 70 -8.4999999999999929];  % mm
  | smiData.RigidTransform(76).angle = 0;  % rad
  | smiData.RigidTransform(76).axis = [0 0 0];
  | smiData.RigidTransform(76).ID = 'AssemblyGround[Bati-1:Assemblage pupitre-1:cavalier_douille_4mm-1]';
  | 
  | %Translation Method - Cartesian
  | %Rotation Method - Arbitrary Axis
  | smiData.RigidTransform(77).translation = [182 70 -8.5];  % mm
  | smiData.RigidTransform(77).angle = 0;  % rad
  | smiData.RigidTransform(77).axis = [0 0 0];
  | smiData.RigidTransform(77).ID = 'AssemblyGround[Bati-1:Assemblage pupitre-1:cavalier_douille_4mm-2]';
  | 
  | %Translation Method - Cartesian
  | %Rotation Method - Arbitrary Axis
  | smiData.RigidTransform(78).translation = [0 0 0];  % mm
  | smiData.RigidTransform(78).angle = 0;  % rad
  | smiData.RigidTransform(78).axis = [0 0 0];
  | smiData.RigidTransform(78).ID = 'AssemblyGround[Bati-1:Assemblage pupitre-1:BP_noir-2:embase_BP_2_contacts-1]';
  | 
  | %Translation Method - Cartesian
  | %Rotation Method - Arbitrary Axis
  | smiData.RigidTransform(79).translation = [15 8.0000000000000071 -20.000000000000018];  % mm
  | smiData.RigidTransform(79).angle = 1.5707963267948968;  % rad
  | smiData.RigidTransform(79).axis = [-1 -0 -0];
  | smiData.RigidTransform(79).ID = 'AssemblyGround[Bati-1:Assemblage pupitre-1:BP_noir-2:corps_BP-3]';
  | 
  | %Translation Method - Cartesian
  | %Rotation Method - Arbitrary Axis
  | smiData.RigidTransform(80).translation = [14.999999999999986 26.000000000000021 -20.000000000000018];  % mm
  | smiData.RigidTransform(80).angle = 1.5707963267948968;  % rad
  | smiData.RigidTransform(80).axis = [-1 -0 -0];
  | smiData.RigidTransform(80).ID = 'AssemblyGround[Bati-1:Assemblage pupitre-1:BP_noir-2:tête_BP_noir-1]';
  | 
  | %Translation Method - Cartesian
  | %Rotation Method - Arbitrary Axis
  | smiData.RigidTransform(81).translation = [22.000000000000007 44.999999999999929 -20.500000000000018];  % mm
  | smiData.RigidTransform(81).angle = 1.5707963267948968;  % rad
  | smiData.RigidTransform(81).axis = [1 0 0];
  | smiData.RigidTransform(81).ID = 'AssemblyGround[Bati-1:Assemblage pupitre-1:BP_noir-2]';
  | 
  | %Translation Method - Cartesian
  | %Rotation Method - Arbitrary Axis
  | smiData.RigidTransform(82).translation = [152.00000000000003 70 -8.5];  % mm
  | smiData.RigidTransform(82).angle = 0;  % rad
  | smiData.RigidTransform(82).axis = [0 0 0];
  | smiData.RigidTransform(82).ID = 'AssemblyGround[Bati-1:Assemblage pupitre-1:cavalier_douille_4mm-3]';
  | 
  | %Translation Method - Cartesian
  | %Rotation Method - Arbitrary Axis
  | smiData.RigidTransform(83).translation = [0 0 0];  % mm
  | smiData.RigidTransform(83).angle = 0;  % rad
  | smiData.RigidTransform(83).axis = [0 0 0];
  | smiData.RigidTransform(83).ID = 'AssemblyGround[Bati-1:Assemblage pupitre-1:BP_noir-1:embase_BP_2_contacts-1]';
  | 
  | %Translation Method - Cartesian
  | %Rotation Method - Arbitrary Axis
  | smiData.RigidTransform(84).translation = [15 8.0000000000000071 -20.000000000000018];  % mm
  | smiData.RigidTransform(84).angle = 1.5707963267948968;  % rad
  | smiData.RigidTransform(84).axis = [-1 -0 -0];
  | smiData.RigidTransform(84).ID = 'AssemblyGround[Bati-1:Assemblage pupitre-1:BP_noir-1:corps_BP-3]';
  | 
  | %Translation Method - Cartesian
  | %Rotation Method - Arbitrary Axis
  | smiData.RigidTransform(85).translation = [14.999999999999986 26.000000000000021 -20.000000000000018];  % mm
  | smiData.RigidTransform(85).angle = 1.5707963267948968;  % rad
  | smiData.RigidTransform(85).axis = [-1 -0 -0];
  | smiData.RigidTransform(85).ID = 'AssemblyGround[Bati-1:Assemblage pupitre-1:BP_noir-1:tête_BP_noir-1]';
  | 
  | %Translation Method - Cartesian
  | %Rotation Method - Arbitrary Axis
  | smiData.RigidTransform(86).translation = [22.000000000000007 145.00000000000003 -20.500000000000018];  % mm
  | smiData.RigidTransform(86).angle = 1.5707963267948968;  % rad
  | smiData.RigidTransform(86).axis = [1 0 0];
  | smiData.RigidTransform(86).ID = 'AssemblyGround[Bati-1:Assemblage pupitre-1:BP_noir-1]';
  | 
  | %Translation Method - Cartesian
  | %Rotation Method - Arbitrary Axis
  | smiData.RigidTransform(87).translation = [-106.99999999999355 50.500000000007987 -429.18631672640487];  % mm
  | smiData.RigidTransform(87).angle = 1.5707963267948968;  % rad
  | smiData.RigidTransform(87).axis = [1 -1.5898819697485813e-14 0];
  | smiData.RigidTransform(87).ID = 'AssemblyGround[Bati-1:Assemblage pupitre-1]';
  | 
  | %Translation Method - Cartesian
  | %Rotation Method - Arbitrary Axis
  | smiData.RigidTransform(88).translation = [-124.99999999999994 21.00000000000006 43.813683273583742];  % mm
  | smiData.RigidTransform(88).angle = 3.1415926535897931;  % rad
  | smiData.RigidTransform(88).axis = [-0.98074665978199183 -0.1952843806515665 -0];
  | smiData.RigidTransform(88).ID = 'AssemblyGround[Bati-1:entretoise base-3]';
  | 
  | %Translation Method - Cartesian
  | %Rotation Method - Arbitrary Axis
  | smiData.RigidTransform(89).translation = [-163.50000000000017 -110.5000000000001 24.813683273583734];  % mm
  | smiData.RigidTransform(89).angle = 1.5707963267948968;  % rad
  | smiData.RigidTransform(89).axis = [1 0 0];
  | smiData.RigidTransform(89).ID = 'AssemblyGround[Bati-1:capot-1]';
  | 
  | %Translation Method - Cartesian
  | %Rotation Method - Arbitrary Axis
  | smiData.RigidTransform(90).translation = [124.99999999999999 229.50000000000014 43.813683273583706];  % mm
  | smiData.RigidTransform(90).angle = 3.1415926535897931;  % rad
  | smiData.RigidTransform(90).axis = [-0.98074665978199194 -0.19528438065156678 -0];
  | smiData.RigidTransform(90).ID = 'AssemblyGround[Bati-1:entretoise base-5]';
  | 
  | %Translation Method - Cartesian
  | %Rotation Method - Arbitrary Axis
  | smiData.RigidTransform(91).translation = [-19.67685219205049 218.00190937854052 74.518455957854741];  % mm
  | smiData.RigidTransform(91).angle = 2.4265819552033245;  % rad
  | smiData.RigidTransform(91).axis = [0.37355742687060095 -0.6559172389981206 0.6559172389981055];
  | smiData.RigidTransform(91).ID = 'AssemblyGround[Bati-1:GOUPILLE FENDUE D3 semi-pliee-1]';
  | 
  | %Translation Method - Cartesian
  | %Rotation Method - Arbitrary Axis
  | smiData.RigidTransform(92).translation = [0 56.240107518936448 92.813683273583749];  % mm
  | smiData.RigidTransform(92).angle = 1.8182270826618918;  % rad
  | smiData.RigidTransform(92).axis = [0.44354426525278196 0.44354426525278268 0.77880483403914424];
  | smiData.RigidTransform(92).ID = 'AssemblyGround[Bati-1:3712-1]';
  | 
  | %Translation Method - Cartesian
  | %Rotation Method - Arbitrary Axis
  | smiData.RigidTransform(93).translation = [-15.999999999999904 -9.9999999999999947 15.000000000002414];  % mm
  | smiData.RigidTransform(93).angle = 0.078455949642202663;  % rad
  | smiData.RigidTransform(93).axis = [1.3280097152925709e-15 3.5463208123511394e-14 1];
  | smiData.RigidTransform(93).ID = 'AssemblyGround[Manivelle-1:ehfr_10-1]';
  | 
  | %Translation Method - Cartesian
  | %Rotation Method - Arbitrary Axis
  | smiData.RigidTransform(94).translation = [79.008796978564519 0 -5.5000000000002967];  % mm
  | smiData.RigidTransform(94).angle = 1.5708903288634597;  % rad
  | smiData.RigidTransform(94).axis = [-0.99990600234935312 -0.0096950107203512947 -0.0096950107203504776];
  | smiData.RigidTransform(94).ID = 'AssemblyGround[Manivelle-1:4074-1]';
  | 
  | %Translation Method - Cartesian
  | %Rotation Method - Arbitrary Axis
  | smiData.RigidTransform(95).translation = [0 -10.000000000000002 0];  % mm
  | smiData.RigidTransform(95).angle = 3.1415926535897931;  % rad
  | smiData.RigidTransform(95).axis = [0.70710678118654935 0 0.70710678118654569];
  | smiData.RigidTransform(95).ID = 'AssemblyGround[Manivelle-1:3775-1]';
  | 
  | %Translation Method - Cartesian
  | %Rotation Method - Arbitrary Axis
  | smiData.RigidTransform(96).translation = [-16.000000000000014 -10.000000000000005 -14.999999999997558];  % mm
  | smiData.RigidTransform(96).angle = 3.1415926535897909;  % rad
  | smiData.RigidTransform(96).axis = [0.77436145486897046 -0.6327435003326477 -1.6337846273434116e-15];
  | smiData.RigidTransform(96).ID = 'AssemblyGround[Manivelle-1:vh_10_40 8-8-1]';
  | 
  | %Translation Method - Cartesian
  | %Rotation Method - Arbitrary Axis
  | smiData.RigidTransform(97).translation = [79.008796978564348 28.500875123966736 -5.5000000000002132];  % mm
  | smiData.RigidTransform(97).angle = 1.8103197986577511;  % rad
  | smiData.RigidTransform(97).axis = [-0.78517615731736834 -0.43789176858005152 -0.43789176858005169];
  | smiData.RigidTransform(97).ID = 'AssemblyGround[Manivelle-1:ehfr_6-1]';
  | 
  | %Translation Method - Cartesian
  | %Rotation Method - Arbitrary Axis
  | smiData.RigidTransform(98).translation = [79.008796978564391 25.000000000000064 -5.5000000000001856];  % mm
  | smiData.RigidTransform(98).angle = 1.6494577526232994;  % rad
  | smiData.RigidTransform(98).axis = [-0.92427773573234051 -0.26991727179776648 -0.26991727179776487];
  | smiData.RigidTransform(98).ID = 'AssemblyGround[Manivelle-1:rond_m_6-1]';
  | 
  | %Translation Method - Cartesian
  | %Rotation Method - Arbitrary Axis
  | smiData.RigidTransform(99).translation = [355.70228863374842 0 0];  % mm
  | smiData.RigidTransform(99).angle = 2.0943951023931957;  % rad
  | smiData.RigidTransform(99).axis = [-0.57735026918962584 0.57735026918962584 -0.57735026918962584];
  | smiData.RigidTransform(99).ID = 'AssemblyGround[Masse_mobile-1:bride-1]';
  | 
  | %Translation Method - Cartesian
  | %Rotation Method - Arbitrary Axis
  | smiData.RigidTransform(100).translation = [255.70228863374845 0 0];  % mm
  | smiData.RigidTransform(100).angle = 2.0943951023931957;  % rad
  | smiData.RigidTransform(100).axis = [-0.57735026918962573 0.57735026918962562 -0.57735026918962595];
  | smiData.RigidTransform(100).ID = 'AssemblyGround[Masse_mobile-1:masse flottante-1]';
  | 
  | %Translation Method - Cartesian
  | %Rotation Method - Arbitrary Axis
  | smiData.RigidTransform(101).translation = [0 -101.00000000000001 0];  % mm
  | smiData.RigidTransform(101).angle = 1.5707963267948959;  % rad
  | smiData.RigidTransform(101).axis = [1 -3.5122758583464524e-23 -5.5834897423476072e-16];
  | smiData.RigidTransform(101).ID = 'AssemblyGround[Bielle-1:3902-1]';
  | 
  | %Translation Method - Cartesian
  | %Rotation Method - Arbitrary Axis
  | smiData.RigidTransform(102).translation = [-3.961376397691124 0 -37.593982191779325];  % mm
  | smiData.RigidTransform(102).angle = 1.7273118015914222;  % rad
  | smiData.RigidTransform(102).axis = [0.85456864553698064 -0.36722774273268793 0.36722774273268793];
  | smiData.RigidTransform(102).ID = 'AssemblyGround[Bielle-1:bielle-1]';
  | 
  | %Translation Method - Cartesian
  | %Rotation Method - Arbitrary Axis
  | smiData.RigidTransform(103).translation = [-42.84115634588715 1.4999999999999458 -2.1983942802717009];  % mm
  | smiData.RigidTransform(103).angle = 1.7273118015914226;  % rad
  | smiData.RigidTransform(103).axis = [0.85456864553698042 -0.36722774273268799 0.36722774273268821];
  | smiData.RigidTransform(103).ID = 'AssemblyGround[Bielle-1:languette-2]';
  | 
  | %Translation Method - Cartesian
  | %Rotation Method - Arbitrary Axis
  | smiData.RigidTransform(104).translation = [0 -410.00000000000006 0];  % mm
  | smiData.RigidTransform(104).angle = 2.0943951023931953;  % rad
  | smiData.RigidTransform(104).axis = [-0.57735026918962584 0.57735026918962584 0.57735026918962562];
  | smiData.RigidTransform(104).ID = 'AssemblyGround[Bielle-1:support barriere-1]';
  | 
  | %Translation Method - Cartesian
  | %Rotation Method - Arbitrary Axis
  | smiData.RigidTransform(105).translation = [-26.695739790461417 0 4.6496582645038229];  % mm
  | smiData.RigidTransform(105).angle = 1.7273118015914224;  % rad
  | smiData.RigidTransform(105).axis = [0.85456864553698031 -0.36722774273268821 0.36722774273268821];
  | smiData.RigidTransform(105).ID = 'AssemblyGround[Bielle-1:butée1-1]';
  | 
  | %Translation Method - Cartesian
  | %Rotation Method - Arbitrary Axis
  | smiData.RigidTransform(106).translation = [940.00000000000057 0 0];  % mm
  | smiData.RigidTransform(106).angle = 2.0943951023931953;  % rad
  | smiData.RigidTransform(106).axis = [-0.57735026918962584 -0.57735026918962584 0.57735026918962584];
  | smiData.RigidTransform(106).ID = 'AssemblyGround[Bielle-1:lisse-1:masse exterieure-1]';
  | 
  | %Translation Method - Cartesian
  | %Rotation Method - Arbitrary Axis
  | smiData.RigidTransform(107).translation = [0 0 0];  % mm
  | smiData.RigidTransform(107).angle = 0;  % rad
  | smiData.RigidTransform(107).axis = [0 0 0];
  | smiData.RigidTransform(107).ID = 'AssemblyGround[Bielle-1:lisse-1:lisse1-1]';
  | 
  | %Translation Method - Cartesian
  | %Rotation Method - Arbitrary Axis
  | smiData.RigidTransform(108).translation = [45.000000000000036 -416.00000000000006 0];  % mm
  | smiData.RigidTransform(108).angle = 3.1415926535897931;  % rad
  | smiData.RigidTransform(108).axis = [8.4285805368518407e-17 1 -2.1131021721274176e-16];
  | smiData.RigidTransform(108).ID = 'AssemblyGround[Bielle-1:lisse-1]';
  | 
  | %Translation Method - Cartesian
  | %Rotation Method - Arbitrary Axis
  | smiData.RigidTransform(109).translation = [-42.841156345887143 -15.000000000000048 -2.1983942802716872];  % mm
  | smiData.RigidTransform(109).angle = 1.7273118015914228;  % rad
  | smiData.RigidTransform(109).axis = [0.8545686455369802 -0.36722774273268827 0.36722774273268843];
  | smiData.RigidTransform(109).ID = 'AssemblyGround[Bielle-1:languette-1]';
  | 
  | %Translation Method - Cartesian
  | %Rotation Method - Arbitrary Axis
  | smiData.RigidTransform(110).translation = [-30.339203965001193 -268.00000000000028 -2.9210790420670789];  % mm
  | smiData.RigidTransform(110).angle = 3.1202733663317019;  % rad
  | smiData.RigidTransform(110).axis = [-0.39480876007397792 -0.0045808668053255114 0.91875190265281081];
  | smiData.RigidTransform(110).ID = 'AssemblyGround[Bielle-1:vchc_10_40 8-8-1]';
  | 
  | %Translation Method - Cartesian
  | %Rotation Method - Arbitrary Axis
  | smiData.RigidTransform(111).translation = [0 -242.99999999999983 0];  % mm
  | smiData.RigidTransform(111).angle = 1.7937595096113965;  % rad
  | smiData.RigidTransform(111).axis = [0.79864892353937578 -0.42553489688238089 0.42553489688237994];
  | smiData.RigidTransform(111).ID = 'AssemblyGround[Bielle-1:3748-1]';
  | 
  | %Translation Method - Cartesian
  | %Rotation Method - Arbitrary Axis
  | smiData.RigidTransform(112).translation = [0 -268 0];  % mm
  | smiData.RigidTransform(112).angle = 1.7273118015914217;  % rad
  | smiData.RigidTransform(112).axis = [0.85456864553698064 -0.36722774273268793 0.36722774273268788];
  | smiData.RigidTransform(112).ID = 'AssemblyGround[Bielle-1:3720-1]';
  | 
  | %Translation Method - Cartesian
  | %Rotation Method - Arbitrary Axis
  | smiData.RigidTransform(113).translation = [-43.399640526413286 3.999999999999948 19.007456219533843];  % mm
  | smiData.RigidTransform(113).angle = 1.6009282379434258;  % rad
  | smiData.RigidTransform(113).axis = [0.97031310413137528 0.17101532087935126 -0.1710153208793512];
  | smiData.RigidTransform(113).ID = 'AssemblyGround[Bielle-1:vis_M3_chcx20-2]';
  | 
  | %Translation Method - Cartesian
  | %Rotation Method - Arbitrary Axis
  | smiData.RigidTransform(114).translation = [0 -399.99999999999994 0];  % mm
  | smiData.RigidTransform(114).angle = 1.8069283767527131;  % rad
  | smiData.RigidTransform(114).axis = [-0.78792093389555207 -0.43541968371282963 -0.43541968371282963];
  | smiData.RigidTransform(114).ID = 'AssemblyGround[Bielle-1:axe-1]';
  | 
  | %Translation Method - Cartesian
  | %Rotation Method - Arbitrary Axis
  | smiData.RigidTransform(115).translation = [-22.752274207133894 3.999999999999948 40.771790899865501];  % mm
  | smiData.RigidTransform(115).angle = 1.7092529506338774;  % rad
  | smiData.RigidTransform(115).axis = [0.8703140719855551 -0.34824805534555531 0.34824805534555542];
  | smiData.RigidTransform(115).ID = 'AssemblyGround[Bielle-1:vis_M3_chcx20-1]';
  | 
  | 
  | %============= Solid =============%
  | %Center of Mass (CoM) %Moments of Inertia (MoI) %Product of Inertia (PoI)
  | 
  | %Initialize the Solid structure array by filling in null values.
  | smiData.Solid(59).mass = 0.0;
  | smiData.Solid(59).CoM = [0.0 0.0 0.0];
  | smiData.Solid(59).MoI = [0.0 0.0 0.0];
  | smiData.Solid(59).PoI = [0.0 0.0 0.0];
  | smiData.Solid(59).color = [0.0 0.0 0.0];
  | smiData.Solid(59).opacity = 0.0;
  | smiData.Solid(59).ID = '';
  | 
  | %Inertia Type - Custom
  | %Visual Properties - Simple
  | smiData.Solid(1).mass = 0.56068208306329503;  % kg
  | smiData.Solid(1).CoM = [0.062086052634561302 -116.53967803560646 11.570309034704412];  % mm
  | smiData.Solid(1).MoI = [5180.1976340359124 5671.3449114845725 10478.486062964139];  % kg*mm^2
  | smiData.Solid(1).PoI = [-520.36303693371258 -1.4296143890206776 -3.9498551615744693];  % kg*mm^2
  | smiData.Solid(1).color = [0.792156862745098 0.81960784313725488 0.93333333333333335];
  | smiData.Solid(1).opacity = 1;
  | smiData.Solid(1).ID = '3742*:*Defaut';
  | 
  | %Inertia Type - Custom
  | %Visual Properties - Simple
  | smiData.Solid(2).mass = 0.0020794911860263017;  % kg
  | smiData.Solid(2).CoM = [-9.373219675548003e-07 0 5.3999999999999986];  % mm
  | smiData.Solid(2).MoI = [0.078738882630271026 0.078738875917678294 0.11988230966518187];  % kg*mm^2
  | smiData.Solid(2).PoI = [4.4898318435102811e-08 0 0];  % kg*mm^2
  | smiData.Solid(2).color = [0.792156862745098 0.81960784313725488 0.93333333333333335];
  | smiData.Solid(2).opacity = 1;
  | smiData.Solid(2).ID = 'eh_12*:*Defaut';
  | 
  | %Inertia Type - Custom
  | %Visual Properties - Simple
  | smiData.Solid(3).mass = 0.00049306016479228152;  % kg
  | smiData.Solid(3).CoM = [-4.2911718685507344e-07 1.2303899426855739e-06 3.7925441961187514];  % mm
  | smiData.Solid(3).MoI = [0.0064238668753637367 0.0064239487949876118 0.0080185339715240535];  % kg*mm^2
  | smiData.Solid(3).PoI = [1.9493093115808118e-09 -6.7449813279502431e-10 4.2726874690727427e-09];  % kg*mm^2
  | smiData.Solid(3).color = [0 0 1];
  | smiData.Solid(3).opacity = 1;
  | smiData.Solid(3).ID = 'ehfr_6*:*Defaut';
  | 
  | %Inertia Type - Custom
  | %Visual Properties - Simple
  | smiData.Solid(4).mass = 1.5257439613510833;  % kg
  | smiData.Solid(4).CoM = [0.096399330707182623 71.957827987059147 -0.096399330707215194];  % mm
  | smiData.Solid(4).MoI = [4331.1083303531495 2392.4099137330618 4331.1083303531495];  % kg*mm^2
  | smiData.Solid(4).PoI = [-12.614628591180844 2.065856679709591 12.614628591184491];  % kg*mm^2
  | smiData.Solid(4).color = [0.792156862745098 0.81960784313725488 0.93333333333333335];
  | smiData.Solid(4).opacity = 1;
  | smiData.Solid(4).ID = 'MOTEUR_014*:*Defaut';
  | 
  | %Inertia Type - Custom
  | %Visual Properties - Simple
  | smiData.Solid(5).mass = 0.0012320066037776716;  % kg
  | smiData.Solid(5).CoM = [-1.1180971344978907e-09 6.8056291294135626e-08 -9.3710780489456962];  % mm
  | smiData.Solid(5).MoI = [0.15264188586060817 0.15264188592086386 0.0093558570497855095];  % kg*mm^2
  | smiData.Solid(5).PoI = [-5.7629862514131982e-10 0 0];  % kg*mm^2
  | smiData.Solid(5).color = [0.792156862745098 0.81960784313725488 0.93333333333333335];
  | smiData.Solid(5).opacity = 1;
  | smiData.Solid(5).ID = 'vchc_6_30*:*Defaut';
  | 
  | %Inertia Type - Custom
  | %Visual Properties - Simple
  | smiData.Solid(6).mass = 0.0044391908260166353;  % kg
  | smiData.Solid(6).CoM = [1.1463772380771852e-07 3.0462694681463573e-06 8.4692956311876486];  % mm
  | smiData.Solid(6).MoI = [0.27502889547007947 0.27503390320514004 0.34199902420956996];  % kg*mm^2
  | smiData.Solid(6).PoI = [6.5063441679595792e-08 -2.3815888135423304e-08 -7.536165454554015e-07];  % kg*mm^2
  | smiData.Solid(6).color = [0.792156862745098 0.81960784313725488 0.93333333333333335];
  | smiData.Solid(6).opacity = 1;
  | smiData.Solid(6).ID = 'ehfr_14*:*Defaut';
  | 
  | %Inertia Type - Custom
  | %Visual Properties - Simple
  | smiData.Solid(7).mass = 0.0020746449565776275;  % kg
  | smiData.Solid(7).CoM = [0 0 1];  % mm
  | smiData.Solid(7).MoI = [0.22307138420346836 0.22307138420346836 0.44476686475975802];  % kg*mm^2
  | smiData.Solid(7).PoI = [0 0 0];  % kg*mm^2
  | smiData.Solid(7).color = [0.792156862745098 0.81960784313725488 0.93333333333333335];
  | smiData.Solid(7).opacity = 1;
  | smiData.Solid(7).ID = 'rond_m_14*:*Defaut';
  | 
  | %Inertia Type - Custom
  | %Visual Properties - Simple
  | smiData.Solid(8).mass = 0.0080690447163568654;  % kg
  | smiData.Solid(8).CoM = [0 19.638622953524315 0];  % mm
  | smiData.Solid(8).MoI = [1.6902866000277663 0.26667857089221397 1.704107222474134];  % kg*mm^2
  | smiData.Solid(8).PoI = [0 -2.1287042035615561e-07 0];  % kg*mm^2
  | smiData.Solid(8).color = [0.792156862745098 0.81960784313725488 0.93333333333333335];
  | smiData.Solid(8).opacity = 1;
  | smiData.Solid(8).ID = 'VIS_TF2E_001*:*Defaut';
  | 
  | %Inertia Type - Custom
  | %Visual Properties - Simple
  | smiData.Solid(9).mass = 0.22329362229061811;  % kg
  | smiData.Solid(9).CoM = [-1.6033091557770751e-05 -0.29550046206916958 29.035335368831966];  % mm
  | smiData.Solid(9).MoI = [148.45697097000229 464.78551406318888 370.29690778425288];  % kg*mm^2
  | smiData.Solid(9).PoI = [0.92173899637463108 0.00011515443130586897 3.5646247255842927e-05];  % kg*mm^2
  | smiData.Solid(9).color = [0.792156862745098 0.81960784313725488 0.93333333333333335];
  | smiData.Solid(9).opacity = 1;
  | smiData.Solid(9).ID = 'roul_010*:*Defaut';
  | 
  | %Inertia Type - Custom
  | %Visual Properties - Simple
  | smiData.Solid(10).mass = 0.00058708512713959236;  % kg
  | smiData.Solid(10).CoM = [0 0 1.0000000000000002];  % mm
  | smiData.Solid(10).MoI = [0.02200040359254879 0.022000403592548786 0.043609417100337847];  % kg*mm^2
  | smiData.Solid(10).PoI = [0 0 0];  % kg*mm^2
  | smiData.Solid(10).color = [0.792156862745098 0.81960784313725488 0.93333333333333335];
  | smiData.Solid(10).opacity = 1;
  | smiData.Solid(10).ID = 'rond_m_10*:*Defaut';
  | 
  | %Inertia Type - Custom
  | %Visual Properties - Simple
  | smiData.Solid(11).mass = 0.0049132603036020836;  % kg
  | smiData.Solid(11).CoM = [-1.2087508164326389e-06 -2.365621925164122e-06 -15.178112071800857];  % mm
  | smiData.Solid(11).MoI = [1.2995970064566389 1.2995969433174015 0.092552857348841749];  % kg*mm^2
  | smiData.Solid(11).PoI = [1.9662991315696181e-07 9.8660146123030184e-08 -9.4144122806409689e-08];  % kg*mm^2
  | smiData.Solid(11).color = [0.792156862745098 0.81960784313725488 0.93333333333333335];
  | smiData.Solid(11).opacity = 1;
  | smiData.Solid(11).ID = 'vh_10_45 8-8*:*Defaut';
  | 
  | %Inertia Type - Custom
  | %Visual Properties - Simple
  | smiData.Solid(12).mass = 0.00093979173435811874;  % kg
  | smiData.Solid(12).CoM = [0 0 3.9999999999999982];  % mm
  | smiData.Solid(12).MoI = [0.025513987771843091 0.025513987771843095 0.041384939360299473];  % kg*mm^2
  | smiData.Solid(12).PoI = [0 0 0];  % kg*mm^2
  | smiData.Solid(12).color = [0.792156862745098 0.81960784313725488 0.93333333333333335];
  | smiData.Solid(12).opacity = 1;
  | smiData.Solid(12).ID = 'ENTRETOISE_023*:*Defaut';
  | 
  | %Inertia Type - Custom
  | %Visual Properties - Simple
  | smiData.Solid(13).mass = 0.1498616086751938;  % kg
  | smiData.Solid(13).CoM = [0 0 12.770120248205542];  % mm
  | smiData.Solid(13).MoI = [69.520182054098299 141.64747697062555 188.18278993969122];  % kg*mm^2
  | smiData.Solid(13).PoI = [0 0 0];  % kg*mm^2
  | smiData.Solid(13).color = [0.792156862745098 0.81960784313725488 0.93333333333333335];
  | smiData.Solid(13).opacity = 1;
  | smiData.Solid(13).ID = 'roul_009*:*Defaut';
  | 
  | %Inertia Type - Custom
  | %Visual Properties - Simple
  | smiData.Solid(14).mass = 0.0019311378596279184;  % kg
  | smiData.Solid(14).CoM = [-6.6731857181254883e-07 2.0172383909890144e-06 6.0111796320415767];  % mm
  | smiData.Solid(14).MoI = [0.064911433236263846 0.064912336270816759 0.082877560400371988];  % kg*mm^2
  | smiData.Solid(14).PoI = [1.9846139203505895e-08 -6.5195431630847546e-09 2.2023837264317799e-07];  % kg*mm^2
  | smiData.Solid(14).color = [0 0 1];
  | smiData.Solid(14).opacity = 1;
  | smiData.Solid(14).ID = 'ehfr_10*:*Defaut';
  | 
  | %Inertia Type - Custom
  | %Visual Properties - Simple
  | smiData.Solid(15).mass = 0.0023561944901923457;  % kg
  | smiData.Solid(15).CoM = [0 0 5];  % mm
  | smiData.Solid(15).MoI = [0.093266031903447025 0.093266031903447025 0.14726215563702161];  % kg*mm^2
  | smiData.Solid(15).PoI = [0 0 0];  % kg*mm^2
  | smiData.Solid(15).color = [0.792156862745098 0.81960784313725488 0.93333333333333335];
  | smiData.Solid(15).opacity = 1;
  | smiData.Solid(15).ID = 'entretoise base*:*Defaut';
  | 
  | %Inertia Type - Custom
  | %Visual Properties - Simple
  | smiData.Solid(16).mass = 0.31810338891001944;  % kg
  | smiData.Solid(16).CoM = [0 172.27503902376517 5];  % mm
  | smiData.Solid(16).MoI = [1441.7751283096197 670.43657814517599 2106.909983306296];  % kg*mm^2
  | smiData.Solid(16).PoI = [0 0 0];  % kg*mm^2
  | smiData.Solid(16).color = [0.792156862745098 0.81960784313725488 0.93333333333333335];
  | smiData.Solid(16).opacity = 1;
  | smiData.Solid(16).ID = 'support moteur*:*Defaut';
  | 
  | %Inertia Type - Custom
  | %Visual Properties - Simple
  | smiData.Solid(17).mass = 0.32787318597035536;  % kg
  | smiData.Solid(17).CoM = [198.14189518515769 1.5 -160.00000000000003];  % mm
  | smiData.Solid(17).MoI = [3023.6361246567326 7701.6013705226951 4678.4570556449171];  % kg*mm^2
  | smiData.Solid(17).PoI = [0 0 0];  % kg*mm^2
  | smiData.Solid(17).color = [0 0 1];
  | smiData.Solid(17).opacity = 1;
  | smiData.Solid(17).ID = 'plateau superieur*:*Defaut';
  | 
  | %Inertia Type - Custom
  | %Visual Properties - Simple
  | smiData.Solid(18).mass = 1.901854999421845;  % kg
  | smiData.Solid(18).CoM = [124.87780167204536 432.38153839200606 -66.975472385051262];  % mm
  | smiData.Solid(18).MoI = [141396.42641440098 25154.306415020677 151943.50584921578];  % kg*mm^2
  | smiData.Solid(18).PoI = [-2787.0294535577987 -1.8649283115950632 -88.866808232734869];  % kg*mm^2
  | smiData.Solid(18).color = [0 0 1];
  | smiData.Solid(18).opacity = 1;
  | smiData.Solid(18).ID = 'base pied*:*Defaut';
  | 
  | %Inertia Type - Custom
  | %Visual Properties - Simple
  | smiData.Solid(19).mass = 1.9371769862953341;  % kg
  | smiData.Solid(19).CoM = [350.00000000000006 4 -175.00000000000003];  % mm
  | smiData.Solid(19).MoI = [19467.912408063996 97009.366617322943 77562.117430446102];  % kg*mm^2
  | smiData.Solid(19).PoI = [0 0 0];  % kg*mm^2
  | smiData.Solid(19).color = [0.75294117647058822 0.75294117647058822 0.75294117647058822];
  | smiData.Solid(19).opacity = 1;
  | smiData.Solid(19).ID = 'socle*:*Defaut';
  | 
  | %Inertia Type - Custom
  | %Visual Properties - Simple
  | smiData.Solid(20).mass = 0.15640000000000004;  % kg
  | smiData.Solid(20).CoM = [67.971014492753611 67.971014492753611 4];  % mm
  | smiData.Solid(20).MoI = [344.3836019323673 344.38360193236701 687.09893719806769];  % kg*mm^2
  | smiData.Solid(20).PoI = [0 0 189.51386473429949];  % kg*mm^2
  | smiData.Solid(20).color = [0 0 1];
  | smiData.Solid(20).opacity = 1;
  | smiData.Solid(20).ID = 'renfort pied*:*Defaut';
  | 
  | %Inertia Type - Custom
  | %Visual Properties - Simple
  | smiData.Solid(21).mass = 0.17667975557891674;  % kg
  | smiData.Solid(21).CoM = [17.984285834740277 33.124791468668612 -40.84525233066497];  % mm
  | smiData.Solid(21).MoI = [152.91768455925404 105.29709625282675 85.644452169266557];  % kg*mm^2
  | smiData.Solid(21).PoI = [-1.8205138347005507 0.035470142853068376 0.11769408986377621];  % kg*mm^2
  | smiData.Solid(21).color = [0.75294117647058822 0.75294117647058822 0.75294117647058822];
  | smiData.Solid(21).opacity = 1;
  | smiData.Solid(21).ID = 'C60*:*Defaut';
  | 
  | %Inertia Type - Custom
  | %Visual Properties - Simple
  | smiData.Solid(22).mass = 0.0017322134258841661;  % kg
  | smiData.Solid(22).CoM = [0 -11.621621061181996 0];  % mm
  | smiData.Solid(22).MoI = [0.098344090649815169 0.035265445630932153 0.098263578130628068];  % kg*mm^2
  | smiData.Solid(22).PoI = [0 0 0];  % kg*mm^2
  | smiData.Solid(22).color = [1 0 0];
  | smiData.Solid(22).opacity = 1;
  | smiData.Solid(22).ID = 'douille_4mm_rouge*:*Defaut';
  | 
  | %Inertia Type - Custom
  | %Visual Properties - Simple
  | smiData.Solid(23).mass = 1.6823036504591504;  % kg
  | smiData.Solid(23).CoM = [52.500000000000007 64.993113833577581 -64.855988039830407];  % mm
  | smiData.Solid(23).MoI = [4579.6221645128708 3830.9072219101731 3617.8922987543115];  % kg*mm^2
  | smiData.Solid(23).PoI = [-0.72570725613490605 0 0];  % kg*mm^2
  | smiData.Solid(23).color = [0.75294117647058822 0.75294117647058822 0.75294117647058822];
  | smiData.Solid(23).opacity = 1;
  | smiData.Solid(23).ID = 'atv*:*Defaut';
  | 
  | %Inertia Type - Custom
  | %Visual Properties - Simple
  | smiData.Solid(24).mass = 0.0091202398229120185;  % kg
  | smiData.Solid(24).CoM = [0 0.96870761480333201 0];  % mm
  | smiData.Solid(24).MoI = [0.62245983488568879 0.76954348407102269 0.62245983488568879];  % kg*mm^2
  | smiData.Solid(24).PoI = [0 0 0];  % kg*mm^2
  | smiData.Solid(24).color = [0.75294117647058822 0.75294117647058822 0.75294117647058822];
  | smiData.Solid(24).opacity = 1;
  | smiData.Solid(24).ID = 'embase_BT_clé*:*Defaut';
  | 
  | %Inertia Type - Custom
  | %Visual Properties - Simple
  | smiData.Solid(25).mass = 0.00041315397343160548;  % kg
  | smiData.Solid(25).CoM = [3.0000000000000022 10.79463824137118 -1.0000000000000009];  % mm
  | smiData.Solid(25).MoI = [0.010914979792664663 0.0066668136156228779 0.017306357425999806];  % kg*mm^2
  | smiData.Solid(25).PoI = [0 0 0];  % kg*mm^2
  | smiData.Solid(25).color = [0.75294117647058822 0.75294117647058822 0.75294117647058822];
  | smiData.Solid(25).opacity = 1;
  | smiData.Solid(25).ID = 'clé*:*Defaut';
  | 
  | %Inertia Type - Custom
  | %Visual Properties - Simple
  | smiData.Solid(26).mass = 0.021600000000000018;  % kg
  | smiData.Solid(26).CoM = [15.000000000000014 -3.7777777777777768 -20.000000000000004];  % mm
  | smiData.Solid(26).MoI = [3.6765333333333374 4.2000000000000091 3.5165333333333395];  % kg*mm^2
  | smiData.Solid(26).PoI = [0 0 0];  % kg*mm^2
  | smiData.Solid(26).color = [0.75294117647058822 0.75294117647058822 0.75294117647058822];
  | smiData.Solid(26).opacity = 1;
  | smiData.Solid(26).ID = 'embase_BP_2_contacts*:*Defaut';
  | 
  | %Inertia Type - Custom
  | %Visual Properties - Simple
  | smiData.Solid(27).mass = 0.0048652566399216782;  % kg
  | smiData.Solid(27).CoM = [2.1024384491229715e-05 5.3820933666692961 4.2284779558526161e-05];  % mm
  | smiData.Solid(27).MoI = [0.21960645461616182 0.34492496167760067 0.21959767846420464];  % kg*mm^2
  | smiData.Solid(27).PoI = [-1.1203197214049224e-06 -1.566800405267401e-06 -5.2154417196044752e-07];  % kg*mm^2
  | smiData.Solid(27).color = [0.75294117647058822 0.75294117647058822 0.75294117647058822];
  | smiData.Solid(27).opacity = 1;
  | smiData.Solid(27).ID = 'corps_BT_clé*:*Defaut';
  | 
  | %Inertia Type - Custom
  | %Visual Properties - Simple
  | smiData.Solid(28).mass = 0.093155640054001232;  % kg
  | smiData.Solid(28).CoM = [104.67905117526601 172.57428557314981 0.75];  % mm
  | smiData.Solid(28).MoI = [1128.2108435862842 429.82613065283749 1558.0020408741018];  % kg*mm^2
  | smiData.Solid(28).PoI = [0 0 12.210751995150186];  % kg*mm^2
  | smiData.Solid(28).color = [0.75294117647058822 0.75294117647058822 0.75294117647058822];
  | smiData.Solid(28).opacity = 1;
  | smiData.Solid(28).ID = 'tole mesures*:*Defaut';
  | 
  | %Inertia Type - Custom
  | %Visual Properties - Simple
  | smiData.Solid(29).mass = 0.0060260328585138734;  % kg
  | smiData.Solid(29).CoM = [0 0 4.9453166577967034];  % mm
  | smiData.Solid(29).MoI = [0.32883055511940029 0.32883055511940024 0.55537822203787957];  % kg*mm^2
  | smiData.Solid(29).PoI = [0 0 0];  % kg*mm^2
  | smiData.Solid(29).color = [0 0.75294117647058822 0];
  | smiData.Solid(29).opacity = 1;
  | smiData.Solid(29).ID = 'tête_voyant_vert*:*Defaut';
  | 
  | %Inertia Type - Custom
  | %Visual Properties - Simple
  | smiData.Solid(30).mass = 0.021966509483079429;  % kg
  | smiData.Solid(30).CoM = [0 0 2.4536279779774737];  % mm
  | smiData.Solid(30).MoI = [4.4338006980672837 3.2754006980672843 3.0639890115594572];  % kg*mm^2
  | smiData.Solid(30).PoI = [0 0 0];  % kg*mm^2
  | smiData.Solid(30).color = [0.75294117647058822 0.75294117647058822 0.75294117647058822];
  | smiData.Solid(30).opacity = 1;
  | smiData.Solid(30).ID = 'corps_voyant_24V*:*Defaut';
  | 
  | %Inertia Type - Custom
  | %Visual Properties - Simple
  | smiData.Solid(31).mass = 0.0037777831702350008;  % kg
  | smiData.Solid(31).CoM = [1.9999999999999991 21.261583343706079 10.492081679318392];  % mm
  | smiData.Solid(31).MoI = [0.68576079147093982 0.1251158900836318 0.58016495294023485];  % kg*mm^2
  | smiData.Solid(31).PoI = [-0.039625411846250146 0 0];  % kg*mm^2
  | smiData.Solid(31).color = [0.75294117647058822 0.75294117647058822 0.75294117647058822];
  | smiData.Solid(31).opacity = 1;
  | smiData.Solid(31).ID = 'inter_sectionneur_vario_4*:*Defaut';
  | 
  | %Inertia Type - Custom
  | %Visual Properties - Simple
  | smiData.Solid(32).mass = 0.033128120998699676;  % kg
  | smiData.Solid(32).CoM = [0 0 0.2594264865308083];  % mm
  | smiData.Solid(32).MoI = [9.259880755376642 9.259880755376642 15.581230810517686];  % kg*mm^2
  | smiData.Solid(32).PoI = [0 0 0];  % kg*mm^2
  | smiData.Solid(32).color = [0.75294117647058822 0.75294117647058822 0.75294117647058822];
  | smiData.Solid(32).opacity = 1;
  | smiData.Solid(32).ID = 'inter_sectionneur_vario_1*:*Defaut';
  | 
  | %Inertia Type - Custom
  | %Visual Properties - Simple
  | smiData.Solid(33).mass = 0.0015662831853071782;  % kg
  | smiData.Solid(33).CoM = [0 0 7.25];  % mm
  | smiData.Solid(33).MoI = [0.40849968068598763 0.40849968068598741 0.81693409957258722];  % kg*mm^2
  | smiData.Solid(33).PoI = [0 0 0];  % kg*mm^2
  | smiData.Solid(33).color = [0.75294117647058822 0.75294117647058822 0.75294117647058822];
  | smiData.Solid(33).opacity = 1;
  | smiData.Solid(33).ID = 'inter_sectionneur_vario_2*:*Defaut';
  | 
  | %Inertia Type - Custom
  | %Visual Properties - Simple
  | smiData.Solid(34).mass = 0.026736590463017754;  % kg
  | smiData.Solid(34).CoM = [-1.0718492961103897e-06 -0.50957986208030015 17.049039568811342];  % mm
  | smiData.Solid(34).MoI = [5.7709195325817655 4.3302739763696101 7.0897276597357886];  % kg*mm^2
  | smiData.Solid(34).PoI = [0.28573504289580887 1.1448832084295697e-07 6.6039191020237154e-05];  % kg*mm^2
  | smiData.Solid(34).color = [1 0 0];
  | smiData.Solid(34).opacity = 1;
  | smiData.Solid(34).ID = 'inter_sectionneur_vario_3*:*Defaut';
  | 
  | %Inertia Type - Custom
  | %Visual Properties - Simple
  | smiData.Solid(35).mass = 0.003425479176304206;  % kg
  | smiData.Solid(35).CoM = [0 9.4999999999999982 19.380166788149808];  % mm
  | smiData.Solid(35).MoI = [0.53590805472747838 0.30762982765655467 0.26868675634217126];  % kg*mm^2
  | smiData.Solid(35).PoI = [0 0 0];  % kg*mm^2
  | smiData.Solid(35).color = [0.75294117647058822 0.75294117647058822 0.75294117647058822];
  | smiData.Solid(35).opacity = 1;
  | smiData.Solid(35).ID = 'cavalier_douille_4mm*:*Defaut';
  | 
  | %Inertia Type - Custom
  | %Visual Properties - Simple
  | smiData.Solid(36).mass = 0.0086539096633947935;  % kg
  | smiData.Solid(36).CoM = [0 0 10.535553841266969];  % mm
  | smiData.Solid(36).MoI = [0.65242919192892823 0.65242919192892834 0.70360148495178987];  % kg*mm^2
  | smiData.Solid(36).PoI = [0 0 0];  % kg*mm^2
  | smiData.Solid(36).color = [0.75294117647058822 0.75294117647058822 0.75294117647058822];
  | smiData.Solid(36).opacity = 1;
  | smiData.Solid(36).ID = 'corps_BP*:*Defaut';
  | 
  | %Inertia Type - Custom
  | %Visual Properties - Simple
  | smiData.Solid(37).mass = 0.0029149398336026566;  % kg
  | smiData.Solid(37).CoM = [0 0 2.9722986645927905];  % mm
  | smiData.Solid(37).MoI = [0.12170606872215252 0.12170606872215249 0.22617182118741064];  % kg*mm^2
  | smiData.Solid(37).PoI = [0 0 0];  % kg*mm^2
  | smiData.Solid(37).color = [0.75294117647058822 0.75294117647058822 0.75294117647058822];
  | smiData.Solid(37).opacity = 1;
  | smiData.Solid(37).ID = 'tête_BP_noir*:*Defaut';
  | 
  | %Inertia Type - Custom
  | %Visual Properties - Simple
  | smiData.Solid(38).mass = 0.5477404149197348;  % kg
  | smiData.Solid(38).CoM = [162.4998154162345 164.07207158532518 -216.48189119172667];  % mm
  | smiData.Solid(38).MoI = [20387.722203457492 23261.742093400124 14980.882195598891];  % kg*mm^2
  | smiData.Solid(38).PoI = [223.87906340590348 0.0060115809507596272 -0.01398493191947445];  % kg*mm^2
  | smiData.Solid(38).color = [1 1 0];
  | smiData.Solid(38).opacity = 1;
  | smiData.Solid(38).ID = 'capot*:*Defaut';
  | 
  | %Inertia Type - Custom
  | %Visual Properties - Simple
  | smiData.Solid(39).mass = 0.00018997881142872628;  % kg
  | smiData.Solid(39).CoM = [8.5901595799028296 0.57598212271217464 0];  % mm
  | smiData.Solid(39).MoI = [0.00080209279889316984 0.008134062277603148 0.0087215030776598874];  % kg*mm^2
  | smiData.Solid(39).PoI = [0 0 -0.00036405534873416411];  % kg*mm^2
  | smiData.Solid(39).color = [0.75294117647058822 0.75294117647058822 0.75294117647058822];
  | smiData.Solid(39).opacity = 1;
  | smiData.Solid(39).ID = 'GOUPILLE FENDUE D3 semi-pliee*:*Defaut';
  | 
  | %Inertia Type - Custom
  | %Visual Properties - Simple
  | smiData.Solid(40).mass = 0.11513955179832987;  % kg
  | smiData.Solid(40).CoM = [53.686357666367094 -2.9656904869068703 0.43065081614338785];  % mm
  | smiData.Solid(40).MoI = [100.2406007548544 253.56071113086821 262.87181303356743];  % kg*mm^2
  | smiData.Solid(40).PoI = [9.7241585980402458 13.373633965757111 -16.116265783205201];  % kg*mm^2
  | smiData.Solid(40).color = [0.792156862745098 0.81960784313725488 0.93333333333333335];
  | smiData.Solid(40).opacity = 1;
  | smiData.Solid(40).ID = '3712*:*Defaut';
  | 
  | %Inertia Type - Custom
  | %Visual Properties - Simple
  | smiData.Solid(41).mass = 0.0055299971876993596;  % kg
  | smiData.Solid(41).CoM = [0 1.8042397414851033e-06 5.9039988411868567];  % mm
  | smiData.Solid(41).MoI = [0.64993019145407638 0.64992974198288445 0.17406971823341069];  % kg*mm^2
  | smiData.Solid(41).PoI = [2.7716264723590607e-08 0 -1.1383150585697625e-08];  % kg*mm^2
  | smiData.Solid(41).color = [0 0 1];
  | smiData.Solid(41).opacity = 1;
  | smiData.Solid(41).ID = '4074*:*Defaut';
  | 
  | %Inertia Type - Custom
  | %Visual Properties - Simple
  | smiData.Solid(42).mass = 0.059334634369084455;  % kg
  | smiData.Solid(42).CoM = [4.9881500926466277e-07 0.066587641376105067 37.510210708090739];  % mm
  | smiData.Solid(42).MoI = [61.905573256748276 64.799911871620225 6.9187844162269254];  % kg*mm^2
  | smiData.Solid(42).PoI = [-0.16752357315292291 0.013694985892205956 1.2435477483283022e-07];  % kg*mm^2
  | smiData.Solid(42).color = [0 0 1];
  | smiData.Solid(42).opacity = 1;
  | smiData.Solid(42).ID = '3775*:*Defaut';
  | 
  | %Inertia Type - Custom
  | %Visual Properties - Simple
  | smiData.Solid(43).mass = 0.004520555945422864;  % kg
  | smiData.Solid(43).CoM = [-1.1995821540976567e-06 -2.3544476819656132e-06 -12.815512406688137];  % mm
  | smiData.Solid(43).MoI = [0.98059530987516208 0.98059525296252492 0.087644018675670607];  % kg*mm^2
  | smiData.Solid(43).PoI = [1.6021154368776186e-07 8.0041564866895952e-08 -8.5949618934549943e-08];  % kg*mm^2
  | smiData.Solid(43).color = [0 0 1];
  | smiData.Solid(43).opacity = 1;
  | smiData.Solid(43).ID = 'vh_10_40 8-8*:*Defaut';
  | 
  | %Inertia Type - Custom
  | %Visual Properties - Simple
  | smiData.Solid(44).mass = 0.00014490596114682917;  % kg
  | smiData.Solid(44).CoM = [0 0 0.60000000000000397];  % mm
  | smiData.Solid(44).MoI = [0.0021751290430396231 0.0021751290430396231 0.004315480655404008];  % kg*mm^2
  | smiData.Solid(44).PoI = [0 0 0];  % kg*mm^2
  | smiData.Solid(44).color = [0 0 1];
  | smiData.Solid(44).opacity = 1;
  | smiData.Solid(44).ID = 'rond_m_6*:*Defaut';
  | 
  | %Inertia Type - Custom
  | %Visual Properties - Simple
  | smiData.Solid(45).mass = 0.0094160513145094219;  % kg
  | smiData.Solid(45).CoM = [0.004093079328754929 -0.009164473299292571 7.4935125115848011];  % mm
  | smiData.Solid(45).MoI = [0.76442472650582627 0.76515245438476043 1.1770054657324862];  % kg*mm^2
  | smiData.Solid(45).PoI = [0.0006046118818123752 -0.00027003454694675102 -0.00040600929404785039];  % kg*mm^2
  | smiData.Solid(45).color = [1 0 0];
  | smiData.Solid(45).opacity = 1;
  | smiData.Solid(45).ID = 'Roue*:*Defaut';
  | 
  | %Inertia Type - Custom
  | %Visual Properties - Simple
  | smiData.Solid(46).mass = 0.06558309099306231;  % kg
  | smiData.Solid(46).CoM = [2.0841569158791646 -0.55527332202158974 9.9652843967183014];  % mm
  | smiData.Solid(46).MoI = [52.72220477401364 46.780028707982169 94.987486758997861];  % kg*mm^2
  | smiData.Solid(46).PoI = [0.0011846364100834411 -0.0040091213830928266 -1.3730124599973883];  % kg*mm^2
  | smiData.Solid(46).color = [0.75294117647058822 0.75294117647058822 0.75294117647058822];
  | smiData.Solid(46).opacity = 1;
  | smiData.Solid(46).ID = 'bride*:*Defaut';
  | 
  | %Inertia Type - Custom
  | %Visual Properties - Simple
  | smiData.Solid(47).mass = 0.35234064403763171;  % kg
  | smiData.Solid(47).CoM = [-0.090278048121520002 0 49.94953499188626];  % mm
  | smiData.Solid(47).MoI = [551.03529131279004 549.83959623149599 515.21356021762801];  % kg*mm^2
  | smiData.Solid(47).PoI = [0 1.1149071191657827 0];  % kg*mm^2
  | smiData.Solid(47).color = [0.75294117647058822 0.75294117647058822 0.75294117647058822];
  | smiData.Solid(47).opacity = 1;
  | smiData.Solid(47).ID = 'masse flottante*:*Defaut';
  | 
  | %Inertia Type - Custom
  | %Visual Properties - Simple
  | smiData.Solid(48).mass = 0.041153292965699521;  % kg
  | smiData.Solid(48).CoM = [0 0 0];  % mm
  | smiData.Solid(48).MoI = [29.646660780435898 29.646660780435898 13.174197910644589];  % kg*mm^2
  | smiData.Solid(48).PoI = [0 0 0];  % kg*mm^2
  | smiData.Solid(48).color = [0.72941176470588232 0.35686274509803922 0.023529411764705882];
  | smiData.Solid(48).opacity = 1;
  | smiData.Solid(48).ID = '3902*:*Defaut';
  | 
  | %Inertia Type - Custom
  | %Visual Properties - Simple
  | smiData.Solid(49).mass = 0.10834827743525144;  % kg
  | smiData.Solid(49).CoM = [30.144438375661842 108.05162927360762 7.5000000700238774];  % mm
  | smiData.Solid(49).MoI = [510.62694656031084 53.836994901956842 560.35596042456712];  % kg*mm^2
  | smiData.Solid(49).PoI = [-3.9449085859211147e-06 3.2649543960993813e-08 0.76687501413309622];  % kg*mm^2
  | smiData.Solid(49).color = [0.72941176470588232 0.35686274509803922 0.023529411764705882];
  | smiData.Solid(49).opacity = 1;
  | smiData.Solid(49).ID = 'bielle*:*Defaut';
  | 
  | %Inertia Type - Custom
  | %Visual Properties - Simple
  | smiData.Solid(50).mass = 0.0018310951377451916;  % kg
  | smiData.Solid(50).CoM = [29.999999999999996 10.355238608479377 0.75];  % mm
  | smiData.Solid(50).MoI = [0.068477595856171206 0.55399769748372196 0.62178863266323869];  % kg*mm^2
  | smiData.Solid(50).PoI = [0 0 0];  % kg*mm^2
  | smiData.Solid(50).color = [0.72941176470588232 0.35686274509803922 0.023529411764705882];
  | smiData.Solid(50).opacity = 1;
  | smiData.Solid(50).ID = 'languette*:*Defaut';
  | 
  | %Inertia Type - Custom
  | %Visual Properties - Simple
  | smiData.Solid(51).mass = 0.15469413677812355;  % kg
  | smiData.Solid(51).CoM = [0 13.880864575287458 50.61048266157529];  % mm
  | smiData.Solid(51).MoI = [408.34819886271805 278.00538419314756 175.47984176859435];  % kg*mm^2
  | smiData.Solid(51).PoI = [87.202416843465983 0 0];  % kg*mm^2
  | smiData.Solid(51).color = [0.72941176470588232 0.35686274509803922 0.023529411764705882];
  | smiData.Solid(51).opacity = 1;
  | smiData.Solid(51).ID = 'support barriere*:*Defaut';
  | 
  | %Inertia Type - Custom
  | %Visual Properties - Simple
  | smiData.Solid(52).mass = 0.0085500000000000003;  % kg
  | smiData.Solid(52).CoM = [15 9.4999999999999982 7.5];  % mm
  | smiData.Solid(52).MoI = [0.41752499999999998 0.80156249999999984 0.89846249999999972];  % kg*mm^2
  | smiData.Solid(52).PoI = [0 0 0];  % kg*mm^2
  | smiData.Solid(52).color = [0.72941176470588232 0.35686274509803922 0.023529411764705882];
  | smiData.Solid(52).opacity = 1;
  | smiData.Solid(52).ID = 'butée1*:*Defaut';
  | 
  | %Inertia Type - Custom
  | %Visual Properties - Simple
  | smiData.Solid(53).mass = 0.27006490230102648;  % kg
  | smiData.Solid(53).CoM = [-6.1693100721850584e-08 -0.026374157963067198 61.229018884095979];  % mm
  | smiData.Solid(53).MoI = [511.21779006358111 511.32313501005854 89.855421953738897];  % kg*mm^2
  | smiData.Solid(53).PoI = [-0.0087878048732219528 1.1117710681788917e-07 2.3118531888806164e-07];  % kg*mm^2
  | smiData.Solid(53).color = [0.75294117647058822 0.75294117647058822 0.75294117647058822];
  | smiData.Solid(53).opacity = 1;
  | smiData.Solid(53).ID = 'masse exterieure*:*Defaut';
  | 
  | %Inertia Type - Custom
  | %Visual Properties - Simple
  | smiData.Solid(54).mass = 0.39852270144681423;  % kg
  | smiData.Solid(54).CoM = [458.35784809459318 -0.49485867263645689 0.0042397238445521408];  % mm
  | smiData.Solid(54).MoI = [329.78418532550478 26136.724678183968 26133.164919145875];  % kg*mm^2
  | smiData.Solid(54).PoI = [0.023822502075466687 -0.79204034380198018 -85.859783411110342];  % kg*mm^2
  | smiData.Solid(54).color = [1 1 1];
  | smiData.Solid(54).opacity = 1;
  | smiData.Solid(54).ID = 'lisse1*:*Defaut';
  | 
  | %Inertia Type - Custom
  | %Visual Properties - Simple
  | smiData.Solid(55).mass = 0.0047853627003247084;  % kg
  | smiData.Solid(55).CoM = [-1.8865037916819686e-09 1.1482762537042319e-07 -11.421735485294844];  % mm
  | smiData.Solid(55).MoI = [1.1338401151188717 1.1338401153457194 0.099825276411995234];  % kg*mm^2
  | smiData.Solid(55).PoI = [-5.0692353548127737e-09 6.9072232268883016e-10 0];  % kg*mm^2
  | smiData.Solid(55).color = [0.72941176470588232 0.35686274509803922 0.023529411764705882];
  | smiData.Solid(55).opacity = 1;
  | smiData.Solid(55).ID = 'vchc_10_40 8-8*:*Defaut';
  | 
  | %Inertia Type - Custom
  | %Visual Properties - Simple
  | smiData.Solid(56).mass = 0.014835024171289509;  % kg
  | smiData.Solid(56).CoM = [2.7468435718623354e-05 -0.27125887447030483 -0.074534092030231369];  % mm
  | smiData.Solid(56).MoI = [3.4576720272373467 3.5314041085436241 4.7441993484503291];  % kg*mm^2
  | smiData.Solid(56).PoI = [0.020426202038947305 1.9383969952488974e-06 -7.5576659736230306e-06];  % kg*mm^2
  | smiData.Solid(56).color = [0.72941176470588232 0.35686274509803922 0.023529411764705882];
  | smiData.Solid(56).opacity = 1;
  | smiData.Solid(56).ID = '3748*:*Defaut';
  | 
  | %Inertia Type - Custom
  | %Visual Properties - Simple
  | smiData.Solid(57).mass = 0.036279034212360686;  % kg
  | smiData.Solid(57).CoM = [9.7329456987984546 0.1856575463144898 0];  % mm
  | smiData.Solid(57).MoI = [7.6090927702905429 18.894590211499093 23.96434228879475];  % kg*mm^2
  | smiData.Solid(57).PoI = [0 0 0.22047198569622278];  % kg*mm^2
  | smiData.Solid(57).color = [0.72941176470588232 0.35686274509803922 0.023529411764705882];
  | smiData.Solid(57).opacity = 1;
  | smiData.Solid(57).ID = '3720*:*Defaut';
  | 
  | %Inertia Type - Custom
  | %Visual Properties - Simple
  | smiData.Solid(58).mass = 0.00020963257465479891;  % kg
  | smiData.Solid(58).CoM = [0 0 10.361117052081864];  % mm
  | smiData.Solid(58).MoI = [0.012468198991732408 0.012468198991732408 0.00046540027669888617];  % kg*mm^2
  | smiData.Solid(58).PoI = [0 0 0];  % kg*mm^2
  | smiData.Solid(58).color = [0.72941176470588232 0.35686274509803922 0.023529411764705882];
  | smiData.Solid(58).opacity = 1;
  | smiData.Solid(58).ID = 'vis_M3_chcx20*:*Defaut';
  | 
  | %Inertia Type - Custom
  | %Visual Properties - Simple
  | smiData.Solid(59).mass = 0.28116055426947029;  % kg
  | smiData.Solid(59).CoM = [0.023721202179788285 -0.055466993429738792 199.97582407544792];  % mm
  | smiData.Solid(59).MoI = [3725.3723075647699 3725.4606527816272 31.532872253175263];  % kg*mm^2
  | smiData.Solid(59).PoI = [-0.59268585320407863 -1.3001729504000996 -0.046084102721740891];  % kg*mm^2
  | smiData.Solid(59).color = [0.72941176470588232 0.35686274509803922 0.023529411764705882];
  | smiData.Solid(59).opacity = 1;
  | smiData.Solid(59).ID = 'axe*:*Defaut';
  | 
  | 
  | %============= Joint =============%
  | %X Revolute Primitive (Rx) %Y Revolute Primitive (Ry) %Z Revolute Primitive (Rz)
  | %X Prismatic Primitive (Px) %Y Prismatic Primitive (Py) %Z Prismatic Primitive (Pz) %Spherical Primitive (S)
  | %Constant Velocity Primitive (CV) %Lead Screw Primitive (LS)
  | %Position Target (Pos)
  | 
  | %Initialize the CylindricalJoint structure array by filling in null values.
  | smiData.CylindricalJoint(1).Rz.Pos = 0.0;
  | smiData.CylindricalJoint(1).Pz.Pos = 0.0;
  | smiData.CylindricalJoint(1).ID = '';
  | 
  | smiData.CylindricalJoint(1).Rz.Pos = -1.8270895618406978e-14;  % deg
  | smiData.CylindricalJoint(1).Pz.Pos = 0;  % mm
  | smiData.CylindricalJoint(1).ID = '[Bielle-1:-:Masse_mobile-1]';
  | 
  | 
  | %Initialize the RevoluteJoint structure array by filling in null values.
  | smiData.RevoluteJoint(3).Rz.Pos = 0.0;
  | smiData.RevoluteJoint(3).ID = '';
  | 
  | smiData.RevoluteJoint(1).Rz.Pos = 126.31675932580075;  % deg
  | smiData.RevoluteJoint(1).ID = '[Bati-1:-:Manivelle-1]';
  | 
  | %This joint has been chosen as a cut joint. Simscape Multibody treats cut joints as algebraic constraints to solve closed kinematic loops. The imported model does not use the state target data for this joint.
  | smiData.RevoluteJoint(2).Rz.Pos = -68.527948561925569;  % deg
  | smiData.RevoluteJoint(2).ID = '[Manivelle-1:-:Roue-1]';
  | 
  | smiData.RevoluteJoint(3).Rz.Pos = 3.2435420769662709e-14;  % deg
  | smiData.RevoluteJoint(3).ID = '[Bati-1:-:Bielle-1]';
undefined symbols (not defined in the file or in its folder): smiData, X, Y, Z
libraries: sm_lib x323, nesl_utility x5
(part 1 of 7)
settings Model: Creator=Renaud  LastModifiedBy=rcostado
settings DataIOCC: ReturnWorkspaceOutputs=on
settings OptimizationCC: LifeSpan=inf
settings DebuggingCC: SFExecutionAtInitializationDiag=none
settings SFSimCC: SimUseLocalCustomCode=on
settings RTWCC: RTWUseLocalCustomCode=on

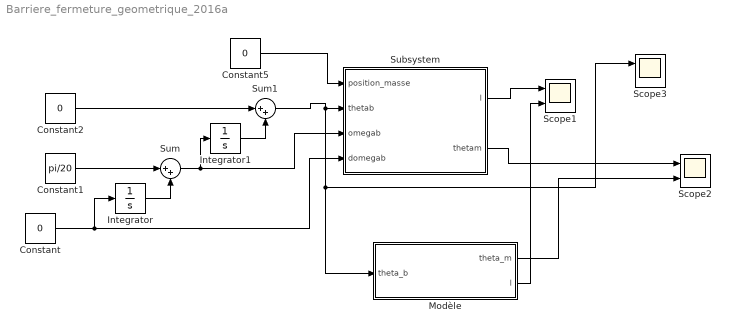
== system Barriere_fermeture_geometrique_2016a ==
  Constant : Constant  Value=0
  Constant1 : Constant  Value=pi/20
  Constant2 : Constant  Value=0
  Constant5 : Constant  Value=0
  Integrator : Integrator
  Integrator1 : Integrator
  Modèle : MATLAB Function  TreatAsAtomicUnit=on
  Scope1 : Scope  NumInputPorts=2
  Scope2 : Scope  NumInputPorts=2
  Scope3 : Scope  NumInputPorts=2
  Subsystem : Subsystem
      mask Display: image('barriere1.png')
  Sum : Sum  Inputs=|++
  Sum1 : Sum  Inputs=|++
  wires:
  Subsystem/1(l) -> Scope1/1
  Subsystem/2(thetam) -> Scope2/1
  Modèle/1(theta_m) -> Scope2/2
  Modèle/2(l) -> Scope1/2
  Integrator1/1 -> Sum1/2
  Constant1/1 -> Sum/1
  Constant2/1 -> Sum1/1
  Integrator/1 -> Sum/2
  Constant/1 -> Subsystem/4(domegab), Integrator/1
  Sum1/1 -> Scope3/1, Modèle/1(theta_b), Subsystem/2(thetab)
  Sum/1 -> Subsystem/3(omegab), Integrator1/1
  Constant5/1 -> Subsystem/1(position_masse)
